simulink model "Automotive_model2"  (R2020b)
settings: Solver=VariableStepAuto  StartTime=0.0  StopTime=97  RelTol=1e-3
undefined symbols (not defined in the file): sigbuilder_block
libraries: simulink x23
(part 1 of 2)
settings Model: Creator=99003757  LastModifiedBy=99003727
settings OptimizationCC: DefaultUnderspecifiedDataType=single
settings DebuggingCC: UniqueDataStoreMsg=error
settings ConfigComp: CovEnable=on  CovScope=ReferencedModels  CovIncludeTopModel=off  CovMetricSettings=dcmwe  CovModelRefEnable=on

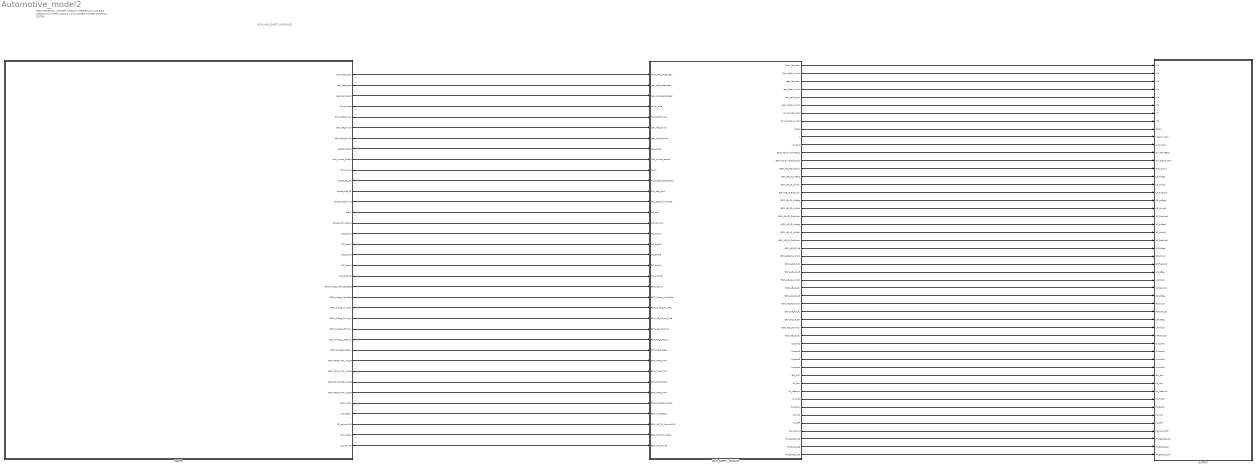
== system Automotive_model2 ==
  note: REQUIREMENTS:
      |
      | 1.POWER WINDOW OPEARTION
      | 2.AIR BAG OPEARTION
      | 3.TPMS
      | 4.DOOR LOCK SYSTEM
      | 5.WIPER CONTROL SYSTEM
  note: BCM_AND_SAFETY_MODULES
  BCM_SAFETY_MODULE : Subsystem
  INPUTS : Subsystem
  OUTPUT : Subsystem
  wires:
  INPUTS/1(Front_left_pass) -> BCM_SAFETY_MODULE/1(Front_left_passenger)
  INPUTS/2(rear_left_pass) -> BCM_SAFETY_MODULE/2(rear_left_passenger)
  INPUTS/3(rear_right_pass) -> BCM_SAFETY_MODULE/3(rear_right_passenger)
  INPUTS/4(Driver_side) -> BCM_SAFETY_MODULE/4(driver_side)
  INPUTS/5(Front_left_driver) -> BCM_SAFETY_MODULE/5(front_left_driver)
  INPUTS/6(rear_left_driver) -> BCM_SAFETY_MODULE/6(rear_left_driver)
  INPUTS/7(rear_right_driver) -> BCM_SAFETY_MODULE/7(rear_right_driver)
  INPUTS/8(object_det_FL) -> BCM_SAFETY_MODULE/8(object_res)
  INPUTS/9(lock_unlock_button) -> BCM_SAFETY_MODULE/9(lock_unlock_control)
  INPUTS/10(ignition_sw) -> BCM_SAFETY_MODULE/10(Ig_sw)
  INPUTS/11(object_det_RL) -> BCM_SAFETY_MODULE/11(Right_left_object_detc)
  INPUTS/12(object_det_RR) -> BCM_SAFETY_MODULE/12(Obj_det_right)
  INPUTS/13(object_det_driver) -> BCM_SAFETY_MODULE/13(Obj_Detc_driver-side)
  INPUTS/14(accln) -> BCM_SAFETY_MODULE/14(DC_Acc)
  INPUTS/15(DC_ignition_status) -> BCM_SAFETY_MODULE/15(DC_iginition)
  INPUTS/16(DC_Door1) -> BCM_SAFETY_MODULE/16(DC_Door1)
  INPUTS/17(DC_Door2) -> BCM_SAFETY_MODULE/17(DC_Door2)
  INPUTS/18(DC_Door3) -> BCM_SAFETY_MODULE/18(DC_Door3)
  INPUTS/19(DC_Door4) -> BCM_SAFETY_MODULE/19(DC_Door4)
  INPUTS/20(DC_antilock) -> BCM_SAFETY_MODULE/20(DC_Antilock)
  INPUTS/21(BAM_Airbag_VehicleSpeed) -> BCM_SAFETY_MODULE/21(BCM_AB_VS)
  INPUTS/22(BCM_Airbag_YawRate) -> BCM_SAFETY_MODULE/22(BCM_Airbag_YawRate)
  INPUTS/23(BCM_Airbag_Air_ACC) -> BCM_SAFETY_MODULE/23(BCM_Airbag_Air_ACC)
  INPUTS/24(BCM_Airbag_Driver_L) -> BCM_SAFETY_MODULE/24(BCM_AB_Driver_Side)
  INPUTS/25(BCM_AirbagL_Front_1) -> BCM_SAFETY_MODULE/25(BCM_AB_L_Front_1)
  INPUTS/26(BCM_Airbag_L_Rear_1) -> BCM_SAFETY_MODULE/26(BCM_AB_L_Rear_1)
  INPUTS/27(BCM_Airbag_R_Rear_) -> BCM_SAFETY_MODULE/27(BCM_AB_R_Rear_)
  BCM_SAFETY_MODULE/1(Front_left_warn) -> OUTPUT/1(In1)
  BCM_SAFETY_MODULE/2(Front_left_window) -> OUTPUT/2(In2)
  BCM_SAFETY_MODULE/3(rear_left_warn) -> OUTPUT/3(In3)
  BCM_SAFETY_MODULE/4(rear_left_window) -> OUTPUT/4(In4)
  BCM_SAFETY_MODULE/5(rear_right_warn) -> OUTPUT/5(In5)
  BCM_SAFETY_MODULE/6(rear_right_window) -> OUTPUT/6(In6)
  BCM_SAFETY_MODULE/7(driver_side_warn) -> OUTPUT/7(In7)
  BCM_SAFETY_MODULE/8(driver_side_window) -> OUTPUT/8(In8)
  BCM_SAFETY_MODULE/9(Delay) -> OUTPUT/9(Delay)
  BCM_SAFETY_MODULE/10(y) -> OUTPUT/10(Interior light)
  BCM_SAFETY_MODULE/11(Outport) -> OUTPUT/11(Automatic)
  BCM_SAFETY_MODULE/12(BCM_AB_DriverAirBag1) -> OUTPUT/12(DriverAirBag1)
  BCM_SAFETY_MODULE/13(BCM_AB_DriverDoorLock) -> OUTPUT/13(DriverDoorLock)
  BCM_SAFETY_MODULE/14(BCM_AB_FuelLock11) -> OUTPUT/14(FuelLock11)
  BCM_SAFETY_MODULE/15(BCM_AB_LF_AirBag) -> OUTPUT/15(LF_AirBag)
  BCM_SAFETY_MODULE/16(BCM_AB_LF_Unlock) -> OUTPUT/16(LF_Unlock)
  BCM_SAFETY_MODULE/17(BCM_AB_LF_FuelLock) -> OUTPUT/17(LF_FuleLock)
  BCM_SAFETY_MODULE/18(BCM_AB_RR_AirBag) -> OUTPUT/18(RR_AirBag)
  BCM_SAFETY_MODULE/19(BCM_AB_RR_Unlock) -> OUTPUT/19(RR_Unlock)
  BCM_SAFETY_MODULE/20(BCM_AB_RR_FuelLock) -> OUTPUT/20(RR_FuelLock)
  BCM_SAFETY_MODULE/21(BCM_AB_LR_AirBag) -> OUTPUT/21(LR_AirBag)
  BCM_SAFETY_MODULE/22(BCM_AB_LR_Unlock) -> OUTPUT/22(LR_Unlock)
  BCM_SAFETY_MODULE/23(BCM_AB_LR_FuelLock) -> OUTPUT/23(LR_FuelLock)
  BCM_SAFETY_MODULE/24(BCM_AB_DS_AB) -> OUTPUT/24(DSAirBag)
  BCM_SAFETY_MODULE/25(BCM_AB_DS_Unlock) -> OUTPUT/25(DSUnlock)
  BCM_SAFETY_MODULE/26(BCM_AB_DS_FL) -> OUTPUT/26(DSFuelLock)
  BCM_SAFETY_MODULE/27(BCM_AB_LS_AB) -> OUTPUT/27(LSAirBag)
  BCM_SAFETY_MODULE/28(BCM_AB_LS_Unlock) -> OUTPUT/28(LSUnlock)
  BCM_SAFETY_MODULE/29(BCM_AB_LS_FL) -> OUTPUT/29(LSFuelLock)
  BCM_SAFETY_MODULE/30(BCM_AB_RS_AB) -> OUTPUT/30(RSAirBag)
  BCM_SAFETY_MODULE/31(BCM_AB_RSUnlock) -> OUTPUT/31(RSUnlock)
  BCM_SAFETY_MODULE/32(BCM_AB_RS_FL) -> OUTPUT/32(RSFuelLock)
  BCM_SAFETY_MODULE/33(BCM_AB_LR_AB) -> OUTPUT/33(LRAirBag)
  BCM_SAFETY_MODULE/34(BCM_AB_LRUnlock) -> OUTPUT/34(LRUnlock)
  BCM_SAFETY_MODULE/35(BCM_AB_LR_FL) -> OUTPUT/35(LRFuelLock)
  BCM_SAFETY_MODULE/36(Outport1) -> OUTPUT/36(Outport1)
  BCM_SAFETY_MODULE/37(Outport2) -> OUTPUT/37(Outport2)
  BCM_SAFETY_MODULE/38(Outport3) -> OUTPUT/38(Outport3)
  BCM_SAFETY_MODULE/39(Outport4) -> OUTPUT/39(Outport4)
  INPUTS/28(BCM_TPMS_TP1_VALUE) -> BCM_SAFETY_MODULE/28(BCM_TPMS_TP1)
  INPUTS/29(BCM_TPMS_TP2_VALUE) -> BCM_SAFETY_MODULE/29(BCM_TPMS_TP2)
  INPUTS/30(BCM_TPMS_TP3_VALUE) -> BCM_SAFETY_MODULE/30(BCM_TPMS_TP3)
  INPUTS/31(BCM_TPMS_TP4_VALUE) -> BCM_SAFETY_MODULE/31(BCM_TPMS_TP4)
  INPUTS/32(Rear_wiper) -> BCM_SAFETY_MODULE/32(BCM_WC_Rear_Wiper)
  INPUTS/33(WC_status) -> BCM_SAFETY_MODULE/33(BCM_WC_Status)
  INPUTS/34(FC_manualINP) -> BCM_SAFETY_MODULE/34(BCM_WC_FR_ManualINP)
  INPUTS/35(FW_Modes) -> BCM_SAFETY_MODULE/35(BCM_WC_FW_Modes)
  INPUTS/36(WC_FrontS) -> BCM_SAFETY_MODULE/36(BCM_WC_FrontS)
  BCM_SAFETY_MODULE/40(BW_OUT) -> OUTPUT/40(BW_out)
  BCM_SAFETY_MODULE/41(FA_Low) -> OUTPUT/41(FA_Low)
  BCM_SAFETY_MODULE/42(FA_Medium) -> OUTPUT/42(FA_Medium)
  BCM_SAFETY_MODULE/43(FA_High) -> OUTPUT/43(FA_HIGH)
  BCM_SAFETY_MODULE/44(FA_Spray) -> OUTPUT/44(FA_Spray)
  BCM_SAFETY_MODULE/45(FA_Mist) -> OUTPUT/45(FA_Mist)
  BCM_SAFETY_MODULE/46(FA_OFF) -> OUTPUT/46(FA_OFF)
  BCM_SAFETY_MODULE/47(Manual_out) -> OUTPUT/47(Manual_OUT)
  BCM_SAFETY_MODULE/48(FM_lessthan30) -> OUTPUT/48(FM_lessthan30)
  BCM_SAFETY_MODULE/49(FM_Bw30_60) -> OUTPUT/49(FM_Bw30_60)
  BCM_SAFETY_MODULE/50(FM_Bw60_100) -> OUTPUT/50(FM_Bw60_100)

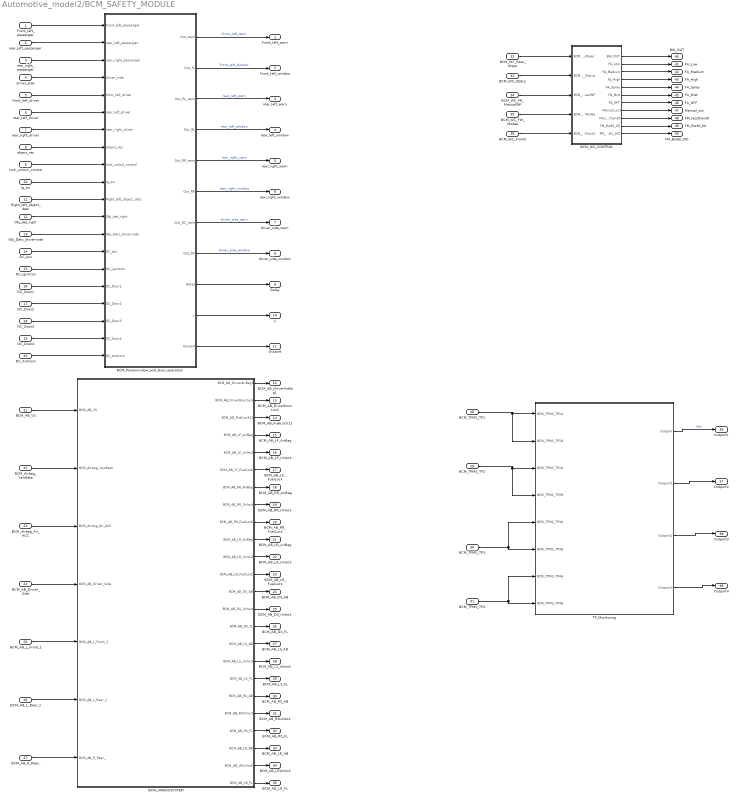
== system Automotive_model2/BCM_SAFETY_MODULE ==
  Front_left_passenger : Inport
  rear_left_passenger : Inport  Port=2
  rear_right_passenger : Inport  Port=3
  driver_side : Inport  Port=4
  front_left_driver : Inport  Port=5
  rear_left_driver : Inport  Port=6
  rear_right_driver : Inport  Port=7
  object_res : Inport  Port=8
  lock_unlock_control : Inport  Port=9
  Ig_sw : Inport  Port=10
  Right_left_object_detc : Inport  Port=11
  Obj_det_right : Inport  Port=12
  Obj_Detc_driver-side : Inport  Port=13
  DC_Acc : Inport  Port=14
  DC_iginition : Inport  Port=15
  DC_Door1 : Inport  Port=16
  DC_Door2 : Inport  Port=17
  DC_Door3 : Inport  Port=18
  DC_Door4 : Inport  Port=19
  DC_Antilock : Inport  Port=20
  BCM_AB_VS : Inport  Port=21
  BCM_Airbag_YawRate : Inport  Port=22
  BCM_Airbag_Air_ACC : Inport  Port=23
  BCM_AB_Driver_Side : Inport  Port=24
  BCM_AB_L_Front_1 : Inport  Port=25
  BCM_AB_L_Rear_1 : Inport  Port=26
  BCM_AB_R_Rear_ : Inport  Port=27
  BCM_TPMS_TP1 : Inport  Port=28
  BCM_TPMS_TP2 : Inport  Port=29
  BCM_TPMS_TP3 : Inport  Port=30
  BCM_TPMS_TP4 : Inport  Port=31
  BCM_WC_Rear_Wiper : Inport  Port=32
  BCM_WC_Status : Inport  Port=33
  BCM_WC_FR_ManualINP : Inport  Port=34
  BCM_WC_FW_Modes : Inport  Port=35
  BCM_WC_FrontS : Inport  Port=36
  BCM_AIRBAGSYSTEM : Subsystem
  BCM_Powerwindow_and_Door_operation : Subsystem
  BCM_WC_CONTROL : Subsystem
  TP_Monitoring : Subsystem
  Front_left_warn : Outport
  Front_left_window : Outport  Port=2
  rear_left_warn : Outport  Port=3
  rear_left_window : Outport  Port=4
  rear_right_warn : Outport  Port=5
  rear_right_window : Outport  Port=6
  driver_side_warn : Outport  Port=7
  driver_side_window : Outport  Port=8
  Delay : Outport  Port=9
  y : Outport  Port=10
  Outport : Outport  Port=11
  BCM_AB_DriverAirBag1 : Outport  Port=12
  BCM_AB_DriverDoorLock : Outport  Port=13
  BCM_AB_FuelLock11 : Outport  Port=14
  BCM_AB_LF_AirBag : Outport  Port=15
  BCM_AB_LF_Unlock : Outport  Port=16
  BCM_AB_LF_FuelLock : Outport  Port=17
  BCM_AB_RR_AirBag : Outport  Port=18
  BCM_AB_RR_Unlock : Outport  Port=19
  BCM_AB_RR_FuelLock : Outport  Port=20
  BCM_AB_LR_AirBag : Outport  Port=21
  BCM_AB_LR_Unlock : Outport  Port=22
  BCM_AB_LR_FuelLock : Outport  Port=23
  BCM_AB_DS_AB : Outport  Port=24
  BCM_AB_DS_Unlock : Outport  Port=25
  BCM_AB_DS_FL : Outport  Port=26
  BCM_AB_LS_AB : Outport  Port=27
  BCM_AB_LS_Unlock : Outport  Port=28
  BCM_AB_LS_FL : Outport  Port=29
  BCM_AB_RS_AB : Outport  Port=30
  BCM_AB_RSUnlock : Outport  Port=31
  BCM_AB_RS_FL : Outport  Port=32
  BCM_AB_LR_AB : Outport  Port=33
  BCM_AB_LRUnlock : Outport  Port=34
  BCM_AB_LR_FL : Outport  Port=35
  Outport1 : Outport  Port=36
  Outport2 : Outport  Port=37
  Outport3 : Outport  Port=38
  Outport4 : Outport  Port=39
  BW_OUT : Outport  Port=40
  FA_Low : Outport  Port=41
  FA_Medium : Outport  Port=42
  FA_High : Outport  Port=43
  FA_Spray : Outport  Port=44
  FA_Mist : Outport  Port=45
  FA_OFF : Outport  Port=46
  Manual_out : Outport  Port=47
  FM_lessthan30 : Outport  Port=48
  FM_Bw30_60 : Outport  Port=49
  FM_Bw60_100 : Outport  Port=50
  wires:
  BCM_Powerwindow_and_Door_operation/5(Out_RR_warn) -> rear_right_warn/1  "rear_right_warn"
  BCM_AB_VS/1 -> BCM_AIRBAGSYSTEM/1(BCM_AB_VS)
  BCM_Powerwindow_and_Door_operation/4(Out_RL) -> rear_left_window/1  "rear_left_window"
  BCM_AIRBAGSYSTEM/22(BCM_AB_LR_AB) -> BCM_AB_LR_AB/1
  BCM_AIRBAGSYSTEM/18(BCM_AB_LS_FL) -> BCM_AB_LS_FL/1
  BCM_AIRBAGSYSTEM/10(BCM_AB_LR_AirBag) -> BCM_AB_LR_AirBag/1
  BCM_AIRBAGSYSTEM/11(BCM_AB_LR_Unlock) -> BCM_AB_LR_Unlock/1
  BCM_Powerwindow_and_Door_operation/10(y) -> y/1
  BCM_Powerwindow_and_Door_operation/9(Delay) -> Delay/1
  BCM_Powerwindow_and_Door_operation/7(Out_DC_warn) -> driver_side_warn/1  "driver_side_warn"
  DC_Door2/1 -> BCM_Powerwindow_and_Door_operation/17(DC_Door2)
  BCM_AB_R_Rear_/1 -> BCM_AIRBAGSYSTEM/7(BCM_AB_R_Rear_)
  DC_Door1/1 -> BCM_Powerwindow_and_Door_operation/16(DC_Door1)
  DC_Door3/1 -> BCM_Powerwindow_and_Door_operation/18(DC_Door3)
  BCM_AIRBAGSYSTEM/23(BCM_AB_LRUnlock) -> BCM_AB_LRUnlock/1
  BCM_AIRBAGSYSTEM/24(BCM_AB_LR_FL) -> BCM_AB_LR_FL/1
  BCM_AIRBAGSYSTEM/9(BCM_AB_RR_FuelLock) -> BCM_AB_RR_FuelLock/1
  BCM_AIRBAGSYSTEM/17(BCM_AB_LS_Unlock) -> BCM_AB_LS_Unlock/1
  BCM_Powerwindow_and_Door_operation/6(Out_RR) -> rear_right_window/1  "rear_right_window"
  BCM_Powerwindow_and_Door_operation/1(Out_warn) -> Front_left_warn/1  "Front_left_warn"
  BCM_Powerwindow_and_Door_operation/8(Out_DC) -> driver_side_window/1  "driver_side_window"
  BCM_Powerwindow_and_Door_operation/2(Out_FL) -> Front_left_window/1  "Front_left_window"
  rear_right_driver/1 -> BCM_Powerwindow_and_Door_operation/7(rear_right_driver)
  BCM_Powerwindow_and_Door_operation/11(Outport) -> Outport/1
  Ig_sw/1 -> BCM_Powerwindow_and_Door_operation/10(Ig_sw)
  object_res/1 -> BCM_Powerwindow_and_Door_operation/8(object_res)
  lock_unlock_control/1 -> BCM_Powerwindow_and_Door_operation/9(lock_unlock_control)
  rear_left_passenger/1 -> BCM_Powerwindow_and_Door_operation/2(rear_left_passenger)
  DC_iginition/1 -> BCM_Powerwindow_and_Door_operation/15(DC_iginition)
  DC_Antilock/1 -> BCM_Powerwindow_and_Door_operation/20(DC_Antilock)
  BCM_Powerwindow_and_Door_operation/3(Out_RL_warn) -> rear_left_warn/1  "rear_left_warn"
  DC_Acc/1 -> BCM_Powerwindow_and_Door_operation/14(DC_Acc)
  BCM_AIRBAGSYSTEM/15(BCM_AB_DS_FL) -> BCM_AB_DS_FL/1
  BCM_AIRBAGSYSTEM/3(BCM_AB_FuelLock11) -> BCM_AB_FuelLock11/1
  BCM_AIRBAGSYSTEM/7(BCM_AB_RR_AirBag) -> BCM_AB_RR_AirBag/1
  BCM_AIRBAGSYSTEM/4(BCM_AB_LF_AirBag) -> BCM_AB_LF_AirBag/1
  BCM_AIRBAGSYSTEM/13(BCM_AB_DS_AB) -> BCM_AB_DS_AB/1
  Obj_det_right/1 -> BCM_Powerwindow_and_Door_operation/12(Obj_det_right)
  Obj_Detc_driver-side/1 -> BCM_Powerwindow_and_Door_operation/13(Obj_Detc_driver-side)
  rear_right_passenger/1 -> BCM_Powerwindow_and_Door_operation/3(rear_right_passenger)
  Right_left_object_detc/1 -> BCM_Powerwindow_and_Door_operation/11(Right_left_object_detc)
  driver_side/1 -> BCM_Powerwindow_and_Door_operation/4(driver_side)
  rear_left_driver/1 -> BCM_Powerwindow_and_Door_operation/6(rear_left_driver)
  front_left_driver/1 -> BCM_Powerwindow_and_Door_operation/5(front_left_driver)
  Front_left_passenger/1 -> BCM_Powerwindow_and_Door_operation/1(Front_left_passenger)
  BCM_AIRBAGSYSTEM/1(BCM_AB_DriverAirBag1) -> BCM_AB_DriverAirBag1/1
  BCM_AIRBAGSYSTEM/5(BCM_AB_LF_Unlock) -> BCM_AB_LF_Unlock/1
  BCM_AIRBAGSYSTEM/8(BCM_AB_RR_Unlock) -> BCM_AB_RR_Unlock/1
  BCM_AIRBAGSYSTEM/21(BCM_AB_RS_FL) -> BCM_AB_RS_FL/1
  BCM_AIRBAGSYSTEM/20(BCM_AB_RSUnlock) -> BCM_AB_RSUnlock/1
  BCM_AIRBAGSYSTEM/12(BCM_AB_LR_FuelLock) -> BCM_AB_LR_FuelLock/1
  BCM_AIRBAGSYSTEM/19(BCM_AB_RS_AB) -> BCM_AB_RS_AB/1
  BCM_AIRBAGSYSTEM/16(BCM_AB_LS_AB) -> BCM_AB_LS_AB/1
  BCM_AIRBAGSYSTEM/2(BCM_AB_DriverDoorLock) -> BCM_AB_DriverDoorLock/1
  BCM_AIRBAGSYSTEM/6(BCM_AB_LF_FuelLock) -> BCM_AB_LF_FuelLock/1
  BCM_AB_L_Rear_1/1 -> BCM_AIRBAGSYSTEM/6(BCM_AB_L_Rear_1)
  DC_Door4/1 -> BCM_Powerwindow_and_Door_operation/19(DC_Door4)
  BCM_AIRBAGSYSTEM/14(BCM_AB_DS_Unlock) -> BCM_AB_DS_Unlock/1
  BCM_AB_L_Front_1/1 -> BCM_AIRBAGSYSTEM/5(BCM_AB_L_Front_1)
  TP_Monitoring/1(Outport) -> Outport1/1  "op1"
  BCM_AB_Driver_Side/1 -> BCM_AIRBAGSYSTEM/4(BCM_AB_Driver_Side)
  BCM_Airbag_YawRate/1 -> BCM_AIRBAGSYSTEM/2(BCM_Airbag_YawRate)
  BCM_Airbag_Air_ACC/1 -> BCM_AIRBAGSYSTEM/3(BCM_Airbag_Air_ACC)
  TP_Monitoring/3(Outport2) -> Outport3/1
  TP_Monitoring/4(Outport3) -> Outport4/1
  TP_Monitoring/2(Outport1) -> Outport2/1
  BCM_TPMS_TP4/1 -> TP_Monitoring/8(BCM_TPMS_TP4B), TP_Monitoring/7(BCM_TPMS_TP4A)
  BCM_TPMS_TP2/1 -> TP_Monitoring/4(BCM_TPMS_TP2B), TP_Monitoring/3(BCM_TPMS_TP2A)
  BCM_TPMS_TP1/1 -> TP_Monitoring/2(BCM_TPMS_TP1B), TP_Monitoring/1(BCM_TPMS_TP1A)
  BCM_TPMS_TP3/1 -> TP_Monitoring/6(BCM_TPMS_TP3B), TP_Monitoring/5(BCM_TPMS_TP3A)
  BCM_WC_CONTROL/7(FA_OFF) -> FA_OFF/1
  BCM_WC_CONTROL/4(FA_High) -> FA_High/1
  BCM_WC_CONTROL/3(FA_Medium) -> FA_Medium/1
  BCM_WC_CONTROL/2(FA_Low) -> FA_Low/1
  BCM_WC_CONTROL/11(FM_Bw60_100) -> FM_Bw60_100/1
  BCM_WC_FrontS/1 -> BCM_WC_CONTROL/5(BCM_WC_FrontS)
  BCM_WC_Rear_Wiper/1 -> BCM_WC_CONTROL/1(BCM_WC_Rear_Wiper)
  BCM_WC_CONTROL/5(FA_Spray) -> FA_Spray/1
  BCM_WC_FW_Modes/1 -> BCM_WC_CONTROL/4(BCM_WC_FW_Modes)
  BCM_WC_CONTROL/9(FM_lessthan30) -> FM_lessthan30/1
  BCM_WC_FR_ManualINP/1 -> BCM_WC_CONTROL/3(BCM_WC_FR_ManualINP)
  BCM_WC_CONTROL/1(BW_OUT) -> BW_OUT/1
  BCM_WC_CONTROL/10(FM_Bw30_60) -> FM_Bw30_60/1
  BCM_WC_CONTROL/6(FA_Mist) -> FA_Mist/1
  BCM_WC_Status/1 -> BCM_WC_CONTROL/2(BCM_WC_Status)
  BCM_WC_CONTROL/8(Manual_out) -> Manual_out/1

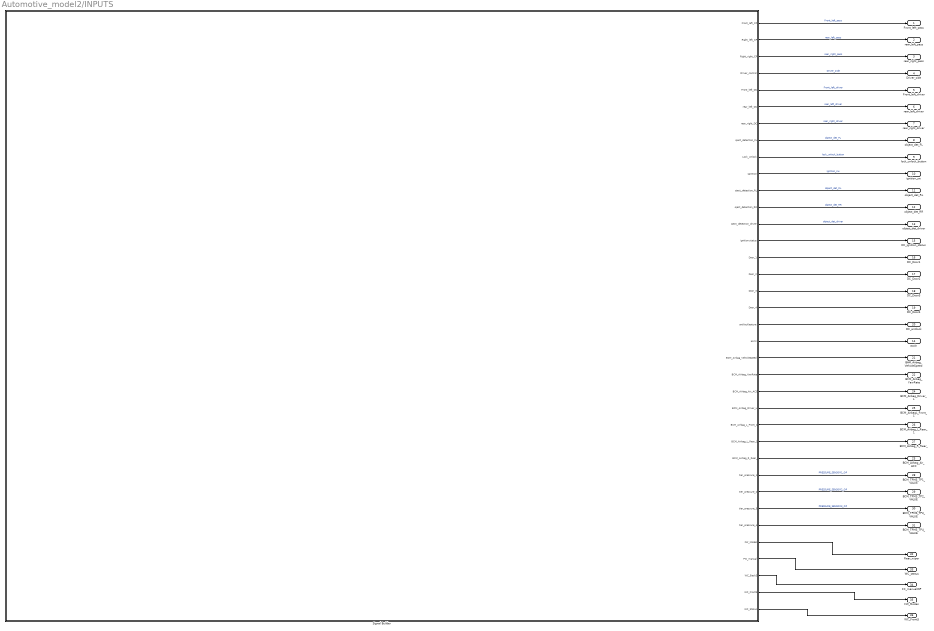
== system Automotive_model2/INPUTS ==
  Signal Builder : Subsystem  Tag=STV Subsys  LoadFcn=sigbuilder_block('load');  StartFcn=sigbuilder_block('start');  StopFcn=sigbuilder_block('stop');  ClipboardFcn=sigbuilder_block('clipboard');  mask(Sigbuilder block){tuvar=[0:10]}
      mask help: Simulink:masks:SigbuilderBlock_MD
      mask init:
      | if ~strcmp(get_param(bdroot(gcbh),'SimulationStatus'),'stopped') tuvar = sigbuilder_block('maskInit'); end
      settings: CopyFcn=sigbuilder_block('copy');  DeleteFcn=sigbuilder_block('delete');  ModelCloseFcn=sigbuilder_block('modelClose');  PreSaveFcn=sigbuilder_block('preSave');  PauseFcn=sigbuilder_block('pause');  ContinueFcn=sigbuilder_block('continue');  NameChangeFcn=sigbuilder_block('namechange');  OpenFcn=sigbuilder_block('open',[6 30 1188 546.75 ]);  CloseFcn=sigbuilder_block('close');
      mask Display: plot(0, 0, 100, 100,[2, 2, 32, 32, 2], [68, 8, 8, 68, 68],[32, 2], [38, 38], [32, 19, 2],[53, 60, 44], [32, 17, 17, 2],[16, 16, 31, 31]);txt = getActiveGroup(gcbh);text(2, 100, txt,'verticalAlignment', 'top');
  Front_left_pass : Outport
  rear_left_pass : Outport  Port=2
  rear_right_pass : Outport  Port=3
  Driver_side : Outport  Port=4
  Front_left_driver : Outport  Port=5
  rear_left_driver : Outport  Port=6
  rear_right_driver : Outport  Port=7
  object_det_FL : Outport  Port=8
  lock_unlock_button : Outport  Port=9
  ignition_sw : Outport  Port=10
  object_det_RL : Outport  Port=11
  object_det_RR : Outport  Port=12
  object_det_driver : Outport  Port=13
  accln : Outport  Port=14
  DC_ignition_status : Outport  Port=15
  DC_Door1 : Outport  Port=16
  DC_Door2 : Outport  Port=17
  DC_Door3 : Outport  Port=18
  DC_Door4 : Outport  Port=19
  DC_antilock : Outport  Port=20
  BAM_Airbag_VehicleSpeed : Outport  Port=21
  BCM_Airbag_YawRate : Outport  Port=22
  BCM_Airbag_Air_ACC : Outport  Port=23
  BCM_Airbag_Driver_L : Outport  Port=24
  BCM_AirbagL_Front_1 : Outport  Port=25
  BCM_Airbag_L_Rear_1 : Outport  Port=26
  BCM_Airbag_R_Rear_ : Outport  Port=27
  BCM_TPMS_TP1_VALUE : Outport  Port=28
  BCM_TPMS_TP2_VALUE : Outport  Port=29
  BCM_TPMS_TP3_VALUE : Outport  Port=30
  BCM_TPMS_TP4_VALUE : Outport  Port=31
  Rear_wiper : Outport  Port=32
  WC_status : Outport  Port=33
  FC_manualINP : Outport  Port=34
  FW_Modes : Outport  Port=35
  WC_FrontS : Outport  Port=36
  wires:
  Signal Builder/14(ignition status) -> DC_ignition_status/1
  Signal Builder/25(BCM_Airbag_L_Front_1) -> BCM_Airbag_L_Rear_1/1
  Signal Builder/21(BCM_Airbag_VehicleSpeed) -> BAM_Airbag_VehicleSpeed/1
  Signal Builder/22(BCM_Airbag_YawRate) -> BCM_Airbag_YawRate/1
  Signal Builder/11(oject_detection_RL) -> object_det_RL/1  "object_det_RL"
  Signal Builder/12(oject_detection_RR) -> object_det_RR/1  "object_det_RR"
  Signal Builder/27(BCM_Airbag_R_Rear_) -> BCM_Airbag_Air_ACC/1
  Signal Builder/26(BCM_Airbag_L_Rear_1) -> BCM_Airbag_R_Rear_/1
  Signal Builder/24(BCM_Airbag_Driver_L) -> BCM_AirbagL_Front_1/1
  Signal Builder/23(BCM_Airbag_Air_ACC) -> BCM_Airbag_Driver_L/1
  Signal Builder/20(accln) -> accln/1
  Signal Builder/19(antilockleature) -> DC_antilock/1
  Signal Builder/2(Right_left_CP) -> rear_left_pass/1  "rear_left_pass"
  Signal Builder/3(Right_right_CP) -> rear_right_pass/1  "rear_right_pass"
  Signal Builder/18(Door_4) -> DC_Door4/1
  Signal Builder/17(Door_3) -> DC_Door3/1
  Signal Builder/16(Door_2) -> DC_Door2/1
  Signal Builder/15(Door_1) -> DC_Door1/1
  Signal Builder/30(tier_pressure_3) -> BCM_TPMS_TP3_VALUE/1  "PRESSURE_SENSOR3_OP"
  Signal Builder/29(tier_pressure_2) -> BCM_TPMS_TP2_VALUE/1  "PRESSURE_SENSOR2_OP"
  Signal Builder/28(tier_pressure_1) -> BCM_TPMS_TP1_VALUE/1  "PRESSURE_SENSOR1_OP"
  Signal Builder/13(oject_detection_driver) -> object_det_driver/1  "object_det_driver"
  Signal Builder/4(Driver_control) -> Driver_side/1  "Driver_side"
  Signal Builder/8(oject_detection_FL) -> object_det_FL/1  "object_det_FL"
  Signal Builder/5(Front_left_DC) -> Front_left_driver/1  "Front_left_driver"
  Signal Builder/7(rear_right_DC) -> rear_right_driver/1  "rear_right_driver"
  Signal Builder/10(iginition) -> ignition_sw/1  "ignition_sw"
  Signal Builder/1(Front_left_CP) -> Front_left_pass/1  "Front_left_pass"
  Signal Builder/6(rear_left_DC) -> rear_left_driver/1  "rear_left_driver"
  Signal Builder/9(Lock_Unlock) -> lock_unlock_button/1  "lock_unlock_button"
  Signal Builder/31(tier_pressure_4) -> BCM_TPMS_TP4_VALUE/1
  Signal Builder/32(FW_Modes) -> Rear_wiper/1
  Signal Builder/33(FW_manual) -> WC_status/1
  Signal Builder/34(WC_BackS) -> FC_manualINP/1
  Signal Builder/35(WC_FrontS) -> FW_Modes/1
  Signal Builder/36(WC_Status) -> WC_FrontS/1

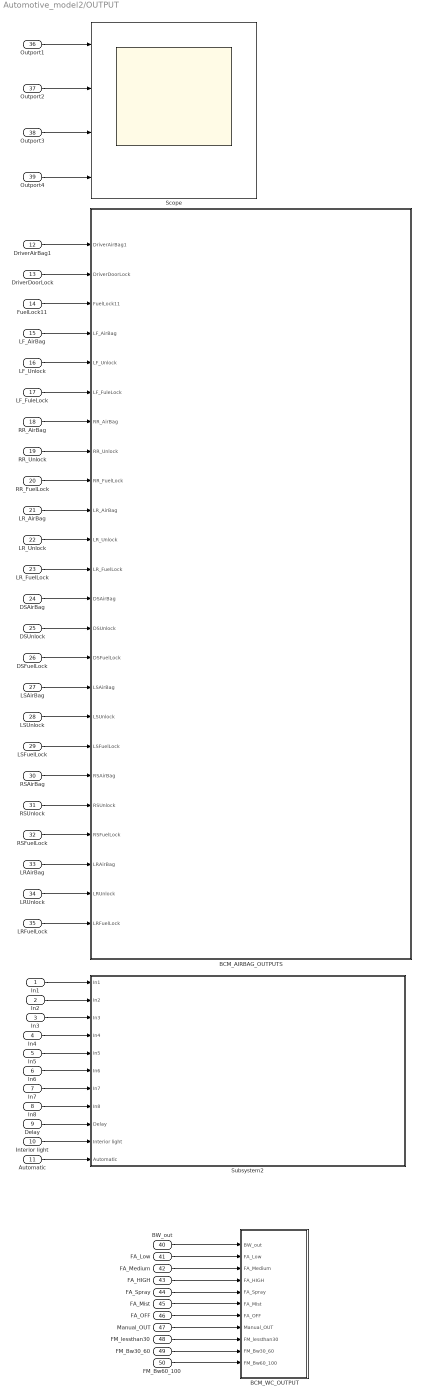
== system Automotive_model2/OUTPUT ==
  In1 : Inport
  In2 : Inport  Port=2
  In3 : Inport  Port=3
  In4 : Inport  Port=4
  In5 : Inport  Port=5
  In6 : Inport  Port=6
  In7 : Inport  Port=7
  In8 : Inport  Port=8
  Delay : Inport  Port=9
  Interior light : Inport  Port=10
  Automatic : Inport  Port=11
  DriverAirBag1 : Inport  Port=12
  DriverDoorLock : Inport  Port=13
  FuelLock11 : Inport  Port=14
  LF_AirBag : Inport  Port=15
  LF_Unlock : Inport  Port=16
  LF_FuleLock : Inport  Port=17
  RR_AirBag : Inport  Port=18
  RR_Unlock : Inport  Port=19
  RR_FuelLock : Inport  Port=20
  LR_AirBag : Inport  Port=21
  LR_Unlock : Inport  Port=22
  LR_FuelLock : Inport  Port=23
  DSAirBag : Inport  Port=24
  DSUnlock : Inport  Port=25
  DSFuelLock : Inport  Port=26
  LSAirBag : Inport  Port=27
  LSUnlock : Inport  Port=28
  LSFuelLock : Inport  Port=29
  RSAirBag : Inport  Port=30
  RSUnlock : Inport  Port=31
  RSFuelLock : Inport  Port=32
  LRAirBag : Inport  Port=33
  LRUnlock : Inport  Port=34
  LRFuelLock : Inport  Port=35
  Outport1 : Inport  Port=36
  Outport2 : Inport  Port=37
  Outport3 : Inport  Port=38
  Outport4 : Inport  Port=39
  BW_out : Inport  Port=40
  FA_Low : Inport  Port=41
  FA_Medium : Inport  Port=42
  FA_HIGH : Inport  Port=43
  FA_Spray : Inport  Port=44
  FA_Mist : Inport  Port=45
  FA_OFF : Inport  Port=46
  Manual_OUT : Inport  Port=47
  FM_lessthan30 : Inport  Port=48
  FM_Bw30_60 : Inport  Port=49
  FM_Bw60_100 : Inport  Port=50
  BCM_AIRBAG_OUTPUTS : Subsystem
  BCM_WC_OUTPUT : Subsystem
  Scope : Scope  NumInputPorts=4
  Subsystem2 : Subsystem
  wires:
  Outport1/1 -> Scope/1
  Outport4/1 -> Scope/4
  Outport3/1 -> Scope/3
  Outport2/1 -> Scope/2
  LSFuelLock/1 -> BCM_AIRBAG_OUTPUTS/18(LSFuelLock)
  RSAirBag/1 -> BCM_AIRBAG_OUTPUTS/19(RSAirBag)
  LRUnlock/1 -> BCM_AIRBAG_OUTPUTS/23(LRUnlock)
  LRAirBag/1 -> BCM_AIRBAG_OUTPUTS/22(LRAirBag)
  RR_FuelLock/1 -> BCM_AIRBAG_OUTPUTS/9(RR_FuelLock)
  LR_Unlock/1 -> BCM_AIRBAG_OUTPUTS/11(LR_Unlock)
  LSUnlock/1 -> BCM_AIRBAG_OUTPUTS/17(LSUnlock)
  LSAirBag/1 -> BCM_AIRBAG_OUTPUTS/16(LSAirBag)
  LR_FuelLock/1 -> BCM_AIRBAG_OUTPUTS/12(LR_FuelLock)
  LR_AirBag/1 -> BCM_AIRBAG_OUTPUTS/10(LR_AirBag)
  DSUnlock/1 -> BCM_AIRBAG_OUTPUTS/14(DSUnlock)
  DSAirBag/1 -> BCM_AIRBAG_OUTPUTS/13(DSAirBag)
  RSFuelLock/1 -> BCM_AIRBAG_OUTPUTS/21(RSFuelLock)
  RSUnlock/1 -> BCM_AIRBAG_OUTPUTS/20(RSUnlock)
  LRFuelLock/1 -> BCM_AIRBAG_OUTPUTS/24(LRFuelLock)
  DSFuelLock/1 -> BCM_AIRBAG_OUTPUTS/15(DSFuelLock)
  RR_AirBag/1 -> BCM_AIRBAG_OUTPUTS/7(RR_AirBag)
  LF_FuleLock/1 -> BCM_AIRBAG_OUTPUTS/6(LF_FuleLock)
  RR_Unlock/1 -> BCM_AIRBAG_OUTPUTS/8(RR_Unlock)
  In7/1 -> Subsystem2/7(In7)
  In4/1 -> Subsystem2/4(In4)
  LF_AirBag/1 -> BCM_AIRBAG_OUTPUTS/4(LF_AirBag)
  LF_Unlock/1 -> BCM_AIRBAG_OUTPUTS/5(LF_Unlock)
  FuelLock11/1 -> BCM_AIRBAG_OUTPUTS/3(FuelLock11)
  DriverAirBag1/1 -> BCM_AIRBAG_OUTPUTS/1(DriverAirBag1)
  Interior light/1 -> Subsystem2/10(Interior light)
  DriverDoorLock/1 -> BCM_AIRBAG_OUTPUTS/2(DriverDoorLock)
  Delay/1 -> Subsystem2/9(Delay)
  In6/1 -> Subsystem2/6(In6)
  Automatic/1 -> Subsystem2/11(Automatic)
  In8/1 -> Subsystem2/8(In8)
  In2/1 -> Subsystem2/2(In2)
  In5/1 -> Subsystem2/5(In5)
  In1/1 -> Subsystem2/1(In1)
  In3/1 -> Subsystem2/3(In3)
  FM_Bw60_100/1 -> BCM_WC_OUTPUT/11(FM_Bw60_100)
  FM_lessthan30/1 -> BCM_WC_OUTPUT/9(FM_lessthan30)
  FA_Mist/1 -> BCM_WC_OUTPUT/6(FA_Mist)
  FA_HIGH/1 -> BCM_WC_OUTPUT/4(FA_HIGH)
  FA_OFF/1 -> BCM_WC_OUTPUT/7(FA_OFF)
  FM_Bw30_60/1 -> BCM_WC_OUTPUT/10(FM_Bw30_60)
  FA_Low/1 -> BCM_WC_OUTPUT/2(FA_Low)
  Manual_OUT/1 -> BCM_WC_OUTPUT/8(Manual_OUT)
  FA_Medium/1 -> BCM_WC_OUTPUT/3(FA_Medium)
  BW_out/1 -> BCM_WC_OUTPUT/1(BW_out)
  FA_Spray/1 -> BCM_WC_OUTPUT/5(FA_Spray)

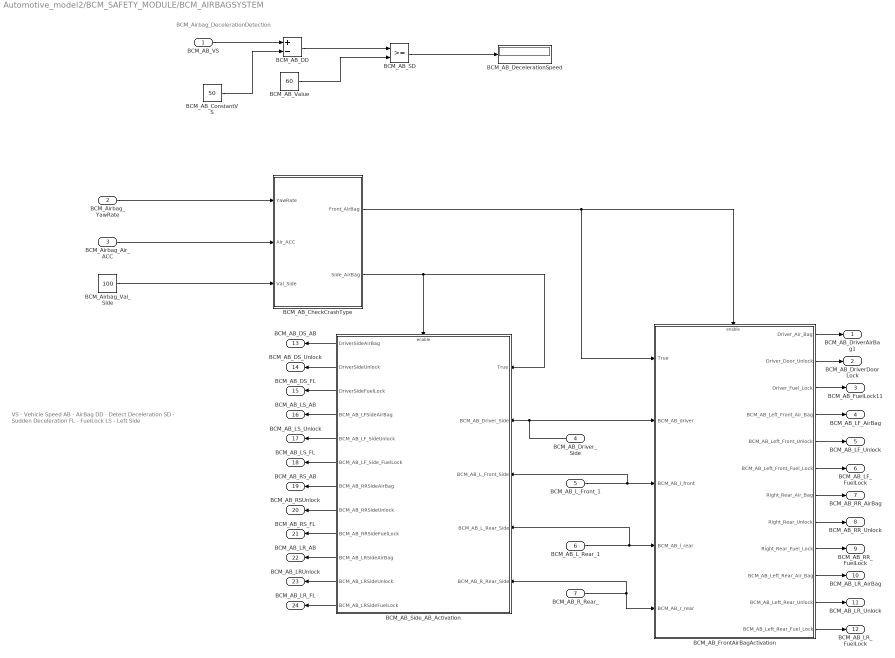
== system Automotive_model2/BCM_SAFETY_MODULE/BCM_AIRBAGSYSTEM ==
  note: VS - Vehicle Speed
      | AB - AirBag
      | DD - Detect Deceleration
      | SD - Sudden Deceleration
      | FL - FuelLock
      | LS - Left Side
  note: BCM_Airbag_DecelerationDetection
  BCM_AB_VS : Inport
  BCM_Airbag_YawRate : Inport  Port=2
  BCM_Airbag_Air_ACC : Inport  Port=3
  BCM_AB_Driver_Side : Inport  Port=4
  BCM_AB_L_Front_1 : Inport  Port=5
  BCM_AB_L_Rear_1 : Inport  Port=6
  BCM_AB_R_Rear_ : Inport  Port=7
  BCM_AB_CheckCrashType : Subsystem
  BCM_AB_ConstantVS : Constant  Value=50
  BCM_AB_DD : Sum  Inputs=+-
  BCM_AB_DecelerationSpeed : Display
  BCM_AB_FrontAirBagActivation : Subsystem  TreatAsAtomicUnit=on
  BCM_AB_SD : RelationalOperator  OutDataTypeStr=boolean  RndMeth=Simplest
  BCM_AB_Side_AB_Activation : Subsystem  TreatAsAtomicUnit=on
  BCM_AB_Value : Constant  Value=60
  BCM_Airbag_Val_Side : Constant  Value=100
  BCM_AB_DriverAirBag1 : Outport
  BCM_AB_DriverDoorLock : Outport  Port=2
  BCM_AB_FuelLock11 : Outport  Port=3
  BCM_AB_LF_AirBag : Outport  Port=4
  BCM_AB_LF_Unlock : Outport  Port=5
  BCM_AB_LF_FuelLock : Outport  Port=6
  BCM_AB_RR_AirBag : Outport  Port=7
  BCM_AB_RR_Unlock : Outport  Port=8
  BCM_AB_RR_FuelLock : Outport  Port=9
  BCM_AB_LR_AirBag : Outport  Port=10
  BCM_AB_LR_Unlock : Outport  Port=11
  BCM_AB_LR_FuelLock : Outport  Port=12
  BCM_AB_DS_AB : Outport  Port=13
  BCM_AB_DS_Unlock : Outport  Port=14
  BCM_AB_DS_FL : Outport  Port=15
  BCM_AB_LS_AB : Outport  Port=16
  BCM_AB_LS_Unlock : Outport  Port=17
  BCM_AB_LS_FL : Outport  Port=18
  BCM_AB_RS_AB : Outport  Port=19
  BCM_AB_RSUnlock : Outport  Port=20
  BCM_AB_RS_FL : Outport  Port=21
  BCM_AB_LR_AB : Outport  Port=22
  BCM_AB_LRUnlock : Outport  Port=23
  BCM_AB_LR_FL : Outport  Port=24
  wires:
  BCM_AB_ConstantVS/1 -> BCM_AB_DD/2
  BCM_AB_Value/1 -> BCM_AB_SD/2
  BCM_AB_DD/1 -> BCM_AB_SD/1
  BCM_AB_SD/1 -> BCM_AB_DecelerationSpeed/1
  BCM_AB_R_Rear_/1 -> BCM_AB_Side_AB_Activation/5(BCM_AB_R_Rear_Side), BCM_AB_FrontAirBagActivation/5(BCM_AB_r_rear)
  BCM_AB_L_Rear_1/1 -> BCM_AB_Side_AB_Activation/4(BCM_AB_L_Rear_Side), BCM_AB_FrontAirBagActivation/4(BCM_AB_l_rear)
  BCM_AB_VS/1 -> BCM_AB_DD/1
  BCM_AB_CheckCrashType/1(Front_AirBag) -> BCM_AB_FrontAirBagActivation/Enable, BCM_AB_FrontAirBagActivation/1(True)
  BCM_AB_CheckCrashType/2(Side_AirBag) -> BCM_AB_Side_AB_Activation/1(True), BCM_AB_Side_AB_Activation/Enable
  BCM_Airbag_YawRate/1 -> BCM_AB_CheckCrashType/1(YawRate)
  BCM_Airbag_Air_ACC/1 -> BCM_AB_CheckCrashType/2(Air_ACC)
  BCM_Airbag_Val_Side/1 -> BCM_AB_CheckCrashType/3(Val_Side)
  BCM_AB_Driver_Side/1 -> BCM_AB_Side_AB_Activation/2(BCM_AB_Driver_Side), BCM_AB_FrontAirBagActivation/2(BCM_AB_driver)
  BCM_AB_L_Front_1/1 -> BCM_AB_Side_AB_Activation/3(BCM_AB_L_Front_Side), BCM_AB_FrontAirBagActivation/3(BCM_AB_l_front)
  BCM_AB_Side_AB_Activation/2(DriverSideUnlock) -> BCM_AB_DS_Unlock/1
  BCM_AB_Side_AB_Activation/3(DriverSideFuelLock) -> BCM_AB_DS_FL/1
  BCM_AB_Side_AB_Activation/1(DriverSideAirBag) -> BCM_AB_DS_AB/1
  BCM_AB_Side_AB_Activation/12(BCM_AB_LRSideFuelLock) -> BCM_AB_LR_FL/1
  BCM_AB_Side_AB_Activation/11(BCM_AB_LRSideUnlock) -> BCM_AB_LRUnlock/1
  BCM_AB_Side_AB_Activation/10(BCM_AB_LRSideAirBag) -> BCM_AB_LR_AB/1
  BCM_AB_Side_AB_Activation/9(BCM_AB_RRSideFuelLock) -> BCM_AB_RS_FL/1
  BCM_AB_Side_AB_Activation/4(BCM_AB_LFSideAirBag) -> BCM_AB_LS_AB/1
  BCM_AB_Side_AB_Activation/5(BCM_AB_LF_SideUnlock) -> BCM_AB_LS_Unlock/1
  BCM_AB_Side_AB_Activation/6(BCM_AB_LF_Side_FuelLock) -> BCM_AB_LS_FL/1
  BCM_AB_Side_AB_Activation/7(BCM_AB_RRSideAirBag) -> BCM_AB_RS_AB/1
  BCM_AB_Side_AB_Activation/8(BCM_AB_RRSideUnlock) -> BCM_AB_RSUnlock/1
  BCM_AB_FrontAirBagActivation/12(BCM_AB_Left_Rear_Fuel_Lock) -> BCM_AB_LR_FuelLock/1
  BCM_AB_FrontAirBagActivation/11(BCM_AB_Left_Rear_Unlock) -> BCM_AB_LR_Unlock/1
  BCM_AB_FrontAirBagActivation/1(Driver_Air_Bag) -> BCM_AB_DriverAirBag1/1
  BCM_AB_FrontAirBagActivation/2(Driver_Door_Unlock) -> BCM_AB_DriverDoorLock/1
  BCM_AB_FrontAirBagActivation/3(Driver_Fuel_Lock) -> BCM_AB_FuelLock11/1
  BCM_AB_FrontAirBagActivation/4(BCM_AB_Left_Front_Air_Bag) -> BCM_AB_LF_AirBag/1
  BCM_AB_FrontAirBagActivation/5(BCM_AB_Left_Front_Unlock) -> BCM_AB_LF_Unlock/1
  BCM_AB_FrontAirBagActivation/6(BCM_AB_Left_Front_Fuel_Lock) -> BCM_AB_LF_FuelLock/1
  BCM_AB_FrontAirBagActivation/7(Right_Rear_Air_Bag) -> BCM_AB_RR_AirBag/1
  BCM_AB_FrontAirBagActivation/8(Right_Rear_Unlock) -> BCM_AB_RR_Unlock/1
  BCM_AB_FrontAirBagActivation/9(Right_Rear_Fuel_Lock) -> BCM_AB_RR_FuelLock/1
  BCM_AB_FrontAirBagActivation/10(BCM_AB_Left_Rear_Air_Bag) -> BCM_AB_LR_AirBag/1

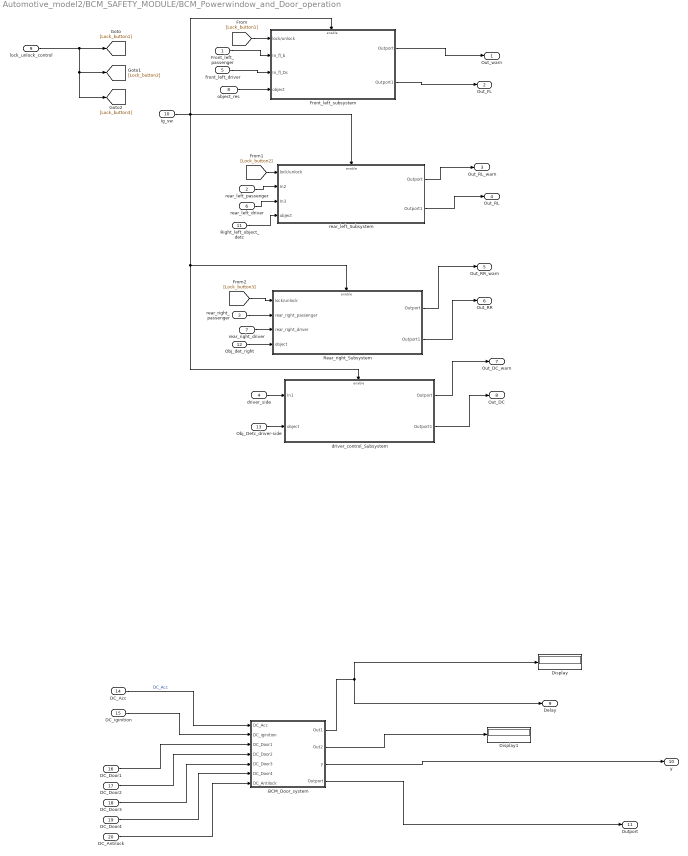
== system Automotive_model2/BCM_SAFETY_MODULE/BCM_Powerwindow_and_Door_operation ==
  Front_left_passenger : Inport
  rear_left_passenger : Inport  Port=2
  rear_right_passenger : Inport  Port=3
  driver_side : Inport  Port=4
  front_left_driver : Inport  Port=5
  rear_left_driver : Inport  Port=6
  rear_right_driver : Inport  Port=7
  object_res : Inport  Port=8
  lock_unlock_control : Inport  Port=9
  Ig_sw : Inport  Port=10
  Right_left_object_detc : Inport  Port=11
  Obj_det_right : Inport  Port=12
  Obj_Detc_driver-side : Inport  Port=13
  DC_Acc : Inport  Port=14
  DC_iginition : Inport  Port=15
  DC_Door1 : Inport  Port=16
  DC_Door2 : Inport  Port=17
  DC_Door3 : Inport  Port=18
  DC_Door4 : Inport  Port=19
  DC_Antilock : Inport  Port=20
  BCM_Door_system : Subsystem
  Display : Display
  Display1 : Display
  Front_left_subsystem : Subsystem
  Rear_right_Subsystem : Subsystem
  driver_control_Subsystem : Subsystem
  rear_left_Subsystem : Subsystem
  Out_warn : Outport
  Out_FL : Outport  Port=2
  Out_RL_warn : Outport  Port=3
  Out_RL : Outport  Port=4
  Out_RR_warn : Outport  Port=5
  Out_RR : Outport  Port=6
  Out_DC_warn : Outport  Port=7
  Out_DC : Outport  Port=8
  Delay : Outport  Port=9
  y : Outport  Port=10
  Outport : Outport  Port=11
  wires:
  Front_left_subsystem/1(Outport) -> Out_warn/1
  Front_left_subsystem/2(Outport1) -> Out_FL/1
  rear_left_Subsystem/1(Outport) -> Out_RL_warn/1
  rear_left_Subsystem/2(Outport1) -> Out_RL/1
  Rear_right_Subsystem/1(Outport) -> Out_RR_warn/1
  Rear_right_Subsystem/2(Outport1) -> Out_RR/1
  driver_control_Subsystem/1(Outport) -> Out_DC_warn/1
  driver_control_Subsystem/2(Outport1) -> Out_DC/1
  lock_unlock_control/1 -> [Lock_button3], [Lock_button2], [Lock_button1]
  front_left_driver/1 -> Front_left_subsystem/3(In_fl_Dc)
  [Lock_button1] -> Front_left_subsystem/1(lock/unlock)
  Front_left_passenger/1 -> Front_left_subsystem/2(In_fl_b)
  rear_left_passenger/1 -> rear_left_Subsystem/2(In2)
  rear_left_driver/1 -> rear_left_Subsystem/3(In3)
  [Lock_button2] -> rear_left_Subsystem/1(lock/unlock)
  rear_right_driver/1 -> Rear_right_Subsystem/3(rear_right_driver)
  rear_right_passenger/1 -> Rear_right_Subsystem/2(rear_right_passenger)
  [Lock_button3] -> Rear_right_Subsystem/1(lock/unlock)
  driver_side/1 -> driver_control_Subsystem/1(In1)
  Ig_sw/1 -> driver_control_Subsystem/Enable, Rear_right_Subsystem/Enable, rear_left_Subsystem/Enable, Front_left_subsystem/Enable
  object_res/1 -> Front_left_subsystem/4(object)
  Right_left_object_detc/1 -> rear_left_Subsystem/4(object)
  Obj_det_right/1 -> Rear_right_Subsystem/4(object)
  Obj_Detc_driver-side/1 -> driver_control_Subsystem/2(object)
  BCM_Door_system/1(Out1) -> Delay/1, Display/1
  DC_Acc/1 -> BCM_Door_system/1(DC_Acc)  "DC_Acc"
  DC_iginition/1 -> BCM_Door_system/2(DC_iginition)
  DC_Door1/1 -> BCM_Door_system/3(DC_Door1)
  DC_Door2/1 -> BCM_Door_system/4(DC_Door2)
  DC_Door3/1 -> BCM_Door_system/5(DC_Door3)
  DC_Door4/1 -> BCM_Door_system/6(DC_Door4)
  DC_Antilock/1 -> BCM_Door_system/7(DC_Antilock)
  BCM_Door_system/2(Out2) -> Display1/1
  BCM_Door_system/3(y) -> y/1
  BCM_Door_system/4(Outport) -> Outport/1

== system Automotive_model2/BCM_SAFETY_MODULE/BCM_WC_CONTROL ==
  note: Wiper Enabling Control:
      |
      | Switch between front, Rear and maual mode.
      | Manual control only works for front wiper
      | When user enables front wiper, he will get 6 modes including manual input.
      | WC status is to switch on/off wiper control
      | There are 3 subsystems for rear, front and manual.
  note: Wiper Control
  note: Front_Windshield
  BCM_WC_Rear_Wiper : Inport
  BCM_WC_Status : Inport  Port=2
  BCM_WC_FR_ManualINP : Inport  Port=3
  BCM_WC_FW_Modes : Inport  Port=4
  BCM_WC_FrontS : Inport  Port=5
  BCM_WC_FR_Automodes : Subsystem
  BCM_WC_FR_manual : Subsystem
  BCM_WC_FW_ENABLE : Switch  Criteria=u2 ~= 0
  BCM_WC_FW_Statuscheck : Logic  IconShape=distinctive  AllPortsSameDT=off  OutDataTypeStr=boolean
  BCM_WC_Rear_windshield : Subsystem
  Constant : Constant  Value=7
  BW_OUT : Outport
  FA_Low : Outport  Port=2
  FA_Medium : Outport  Port=3
  FA_High : Outport  Port=4
  FA_Spray : Outport  Port=5
  FA_Mist : Outport  Port=6
  FA_OFF : Outport  Port=7
  Manual_out : Outport  Port=8
  FM_lessthan30 : Outport  Port=9
  FM_Bw30_60 : Outport  Port=10
  FM_Bw60_100 : Outport  Port=11
  wires:
  BCM_WC_Status/1 -> BCM_WC_FW_Statuscheck/2, BCM_WC_Rear_windshield/2(BCM_WC_StatusINP)
  BCM_WC_FrontS/1 -> BCM_WC_FW_Statuscheck/1
  BCM_WC_FW_Statuscheck/1 -> BCM_WC_FW_ENABLE/2
  BCM_WC_FW_Modes/1 -> BCM_WC_FW_ENABLE/1
  BCM_WC_FW_ENABLE/1 -> BCM_WC_FR_Automodes/1(BCM_FR_AUTOMODES), BCM_WC_FR_manual/1(BCM_FRW_Manualmode)
  BCM_WC_Rear_Wiper/1 -> BCM_WC_Rear_windshield/1(BCM_WC_RearWiperINP)
  BCM_WC_Rear_windshield/1(BW_OUT) -> BW_OUT/1
  BCM_WC_FR_ManualINP/1 -> BCM_WC_FR_manual/2(FW_MANUAL)
  BCM_WC_FR_manual/1(BCM_FRM_Out) -> Manual_out/1
  BCM_WC_FR_manual/2(BCM_FRM_OUT1) -> FM_lessthan30/1
  BCM_WC_FR_manual/3(BCM_FRM_Bw30_60) -> FM_Bw30_60/1
  BCM_WC_FR_manual/4(BCM_FRM__Bw60_100) -> FM_Bw60_100/1
  BCM_WC_FR_Automodes/1(BCM_FR_AUTOMODE_LOWout) -> FA_Low/1
  BCM_WC_FR_Automodes/2(BCM_FR_AUTOMODE_OFF) -> FA_OFF/1
  BCM_WC_FR_Automodes/3(BCM_FR_AUTOMODE_Mediumout) -> FA_Medium/1
  BCM_WC_FR_Automodes/4(BCM_FR_AUTOMODE_High) -> FA_High/1
  BCM_WC_FR_Automodes/5(BCM_FR_AUTOMODE_Spray) -> FA_Spray/1
  BCM_WC_FR_Automodes/6(BCM_FR_AUTOMODE_Mist) -> FA_Mist/1
  Constant/1 -> BCM_WC_FW_ENABLE/3

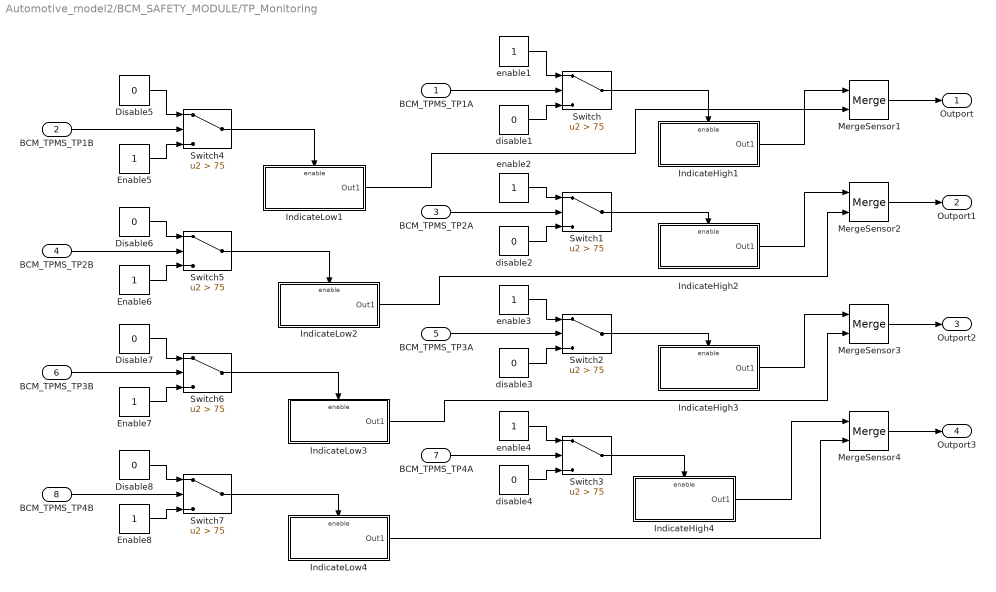
== system Automotive_model2/BCM_SAFETY_MODULE/TP_Monitoring ==
  BCM_TPMS_TP1A : Inport
  BCM_TPMS_TP1B : Inport  Port=2
  BCM_TPMS_TP2A : Inport  Port=3
  BCM_TPMS_TP2B : Inport  Port=4
  BCM_TPMS_TP3A : Inport  Port=5
  BCM_TPMS_TP3B : Inport  Port=6
  BCM_TPMS_TP4A : Inport  Port=7
  BCM_TPMS_TP4B : Inport  Port=8
  Disable{5..8} (4 alike) : Constant  Value=0
  Enable{5..8} (4 alike) : Constant
  IndicateHigh1 : Subsystem  TreatAsAtomicUnit=on
  IndicateHigh2 : Subsystem  TreatAsAtomicUnit=on
  IndicateHigh3 : Subsystem  TreatAsAtomicUnit=on
  IndicateHigh4 : Subsystem  TreatAsAtomicUnit=on
  IndicateLow1 : Subsystem  TreatAsAtomicUnit=on
  IndicateLow2 : Subsystem  TreatAsAtomicUnit=on
  IndicateLow3 : Subsystem  TreatAsAtomicUnit=on
  IndicateLow4 : Subsystem  TreatAsAtomicUnit=on
  MergeSensor{1..4} (4 alike) : Merge
  Switch{,1..7} (8 alike) : Switch  Criteria=u2 > Threshold  Threshold=75
  disable{1..4} (4 alike) : Constant  Value=0
  enable{1..4} (4 alike) : Constant
  Outport : Outport
  Outport1 : Outport  Port=2
  Outport2 : Outport  Port=3
  Outport3 : Outport  Port=4
  wires:
  enable1/1 -> Switch/1
  BCM_TPMS_TP3A/1 -> Switch2/2
  disable1/1 -> Switch/3
  disable3/1 -> Switch2/3
  enable2/1 -> Switch1/1
  BCM_TPMS_TP1A/1 -> Switch/2
  disable4/1 -> Switch3/3
  disable2/1 -> Switch1/3
  enable4/1 -> Switch3/1
  BCM_TPMS_TP2A/1 -> Switch1/2
  BCM_TPMS_TP4A/1 -> Switch3/2
  enable3/1 -> Switch2/1
  Disable8/1 -> Switch7/1
  Enable8/1 -> Switch7/3
  Disable6/1 -> Switch5/1
  Enable6/1 -> Switch5/3
  Enable7/1 -> Switch6/3
  Enable5/1 -> Switch4/3
  Disable5/1 -> Switch4/1
  BCM_TPMS_TP2B/1 -> Switch5/2
  BCM_TPMS_TP3B/1 -> Switch6/2
  BCM_TPMS_TP1B/1 -> Switch4/2
  Disable7/1 -> Switch6/1
  BCM_TPMS_TP4B/1 -> Switch7/2
  Switch3/1 -> IndicateHigh4/Enable
  Switch2/1 -> IndicateHigh3/Enable
  Switch1/1 -> IndicateHigh2/Enable
  Switch/1 -> IndicateHigh1/Enable
  Switch7/1 -> IndicateLow4/Enable
  Switch6/1 -> IndicateLow3/Enable
  Switch5/1 -> IndicateLow2/Enable
  Switch4/1 -> IndicateLow1/Enable
  IndicateHigh1/1(Out1) -> MergeSensor1/1
  IndicateLow1/1(Out1) -> MergeSensor1/2
  IndicateHigh2/1(Out1) -> MergeSensor2/1
  IndicateLow2/1(Out1) -> MergeSensor2/2
  IndicateHigh3/1(Out1) -> MergeSensor3/1
  IndicateLow3/1(Out1) -> MergeSensor3/2
  IndicateHigh4/1(Out1) -> MergeSensor4/1
  IndicateLow4/1(Out1) -> MergeSensor4/2
  MergeSensor1/1 -> Outport/1
  MergeSensor2/1 -> Outport1/1
  MergeSensor3/1 -> Outport2/1
  MergeSensor4/1 -> Outport3/1

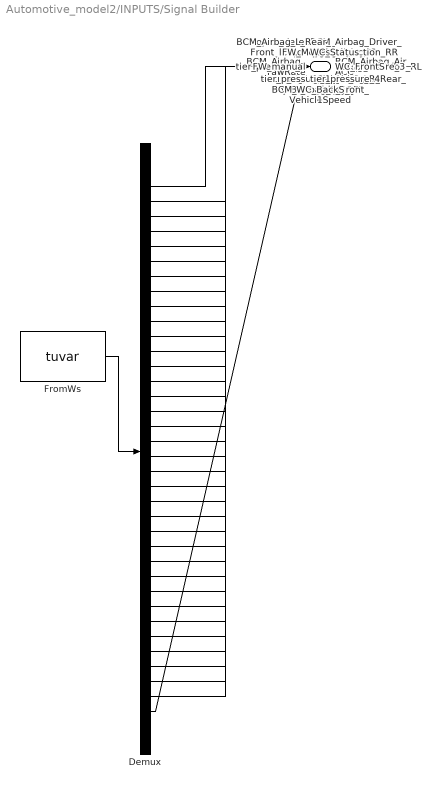
== system Automotive_model2/INPUTS/Signal Builder ==
  Demux : Demux  Tag=STV Demux  Outputs=36
      settings: DisplayOption=none
  FromWs : FromWorkspace  Tag=STV FromWs  VariableName=tuvar
      SigBuilderData=|
      | common.afterFinalStr = 'Extrapolate'
      | common.sampleTime = '0'
      | dataSet.timeRange = [0 97]
      | dataSet.name = 'Sheet1'
      | sbobj.Name = 'Signal Builder'
      | sbobj.Groups.Name = 'Sheet1'
      | sbobj.Groups.Signals(1).Name = 'Front_left_CP'
      | sbobj.Groups.Signals(1).XData = [0 1 2 3 4 5 6 7 8 9 10 11 12 13 14 15 16 17 18 19 20 21 22 23 24 25 26 27 28 29 30 31 32 33 34 35 36 37 38 39 40 41 42 43 44 45 46 47 48 49 50 51 52 53 54 55 56 57 58 59 60 61 62 63 64 65 66 67 68 69 70 71 72 73 74 75 76 77 78 79 80 81 82 83 84 85 86 87 88 89 90 91 92 93 94 95 96 97]
      | sbobj.Groups.Signals(1).YData = [0 0 0 0 0 0 0 1 1 1 1 1 1 1 1 -1 -1 -1 -1 -1 0 1 1 0 -1 -1 1 1 1 0 0 1 1 1 1 0 -1 -1 -1 -1 0 1 1 -1 -1 1 1 1 0 0 0 0 0 0 0 0 1 1 1 1 1 0 0 1 0 0 0 0 0 0 0 0 0 0 0 0 1 1 1 1 -1 -1 1 1 1 0 0 0 0 0 0 0 0 0 0 0 0 0]
      | sbobj.Groups.Signals(2).Name = 'Right_left_CP'
      | sbobj.Groups.Signals(2).XData = [0 1 2 3 4 5 6 7 8 9 10 11 12 13 14 15 16 17 18 19 20 21 22 23 24 25 26 27 28 29 30 31 32 33 34 35 36 37 38 39 40 41 42 43 44 45 46 47 48 49 50 51 52 53 54 55 56 57 58 59 60 61 62 63 64 65 66 67 68 69 70 71 72 73 74 75 76 77 78 79 80 81 82 83 84 85 86 87 88 89 90 91 92 93 94 95 96 97]
      | sbobj.Groups.Signals(2).YData = [0 0 0 0 0 0 0 1 1 1 1 1 1 1 1 -1 -1 -1 -1 -1 0 1 1 0 -1 -1 1 1 1 0 0 1 1 1 1 0 -1 -1 -1 -1 0 1 1 -1 -1 1 1 1 0 0 0 0 0 0 0 0 1 1 1 1 1 0 0 1 0 0 0 0 0 0 0 0 0 0 0 0 1 1 1 1 -1 -1 1 1 1 0 0 0 0 0 0 0 0 0 0 0 0 0]
      | sbobj.Groups.Signals(3).Name = 'Right_right_CP'
      | sbobj.Groups.Signals(3).XData = [0 1 2 3 4 5 6 7 8 9 10 11 12 13 14 15 16 17 18 19 20 21 22 23 24 25 26 27 28 29 30 31 32 33 34 35 36 37 38 39 40 41 42 43 44 45 46 47 48 49 50 51 52 53 54 55 56 57 58 59 60 61 62 63 64 65 66 67 68 69 70 71 72 73 74 75 76 77 78 79 80 81 82 83 84 85 86 87 88 89 90 91 92 93 94 95 96 97]
      | sbobj.Groups.Signals(3).YData = [1 1 0 0 -1 -1 0 1 1 1 1 1 1 1 1 -1 -1 -1 -1 -1 0 1 1 0 -1 -1 1 1 1 0 0 1 1 1 1 0 -1 -1 -1 -1 0 1 1 -1 -1 1 1 1 0 0 0 0 0 0 0 0 1 1 1 1 1 0 0 1 0 0 0 0 0 0 0 0 0 0 0 0 1 1 1 1 -1 -1 1 1 1 0 0 0 0 0 0 0 0 0 0 0 0 0]
      | sbobj.Groups.Signals(4).Name = 'Driver_control'
      | sbobj.Groups.Signals(4).XData = [0 1 2 3 4 5 6 7 8 9 10 11 12 13 14 15 16 17 18 19 20 21 22 23 24 25 26 27 28 29 30 31 32 33 34 35 36 37 38 39 40 41 42 43 44 45 46 47 48 49 50 51 52 53 54 55 56 57 58 59 60 61 62 63 64 65 66 67 68 69 70 71 72 73 74 75 76 77 78 79 80 81 82 83 84 85 86 87 88 89 90 91 92 93 94 95 96 97]
      | sbobj.Groups.Signals(4).YData = [0 0 0 0 0 0 0 1 1 1 1 1 1 1 1 -1 -1 -1 -1 -1 0 1 1 0 -1 -1 1 1 1 1 1 1 1 1 -1 -1 -1 -1 0 1 1 -1 -1 1 1 1 1 1 0 0 0 0 0 0 0 0 1 1 1 1 1 0 0 1 0 0 0 0 0 0 0 0 0 0 0 0 1 1 1 -1 1 1 1 1 1 0 0 0 0 0 0 0 0 0 0 0 0 0]
      | sbobj.Groups.Signals(5).Name = 'Front_left_DC'
      | sbobj.Groups.Signals(5).XData = [0 1 2 3 4 5 6 7 8 9 10 11 12 13 14 15 16 17 18 19 20 21 22 23 24 25 26 27 28 29 30 31 32 33 34 35 36 37 38 39 40 41 42 43 44 45 46 47 48 49 50 51 52 53 54 55 56 57 58 59 60 61 62 63 64 65 66 67 68 69 70 71 72 73 74 75 76 77 78 79 80 81 82 83 84 85 86 87 88 89 90 91 92 93 94 95 96 97]
      | sbobj.Groups.Signals(5).YData = [0 0 0 -1 1 0 0 1 1 1 1 1 1 1 0 -1 -1 -1 -1 -1 0 1 1 0 -1 -1 1 1 1 1 1 -1 0 1 0 0 0 0 0 0 0 0 0 0 0 1 1 1 0 0 0 0 0 0 0 0 1 1 1 1 1 0 0 1 0 0 0 0 0 0 0 0 0 0 0 0 1 1 1 0 0 0 1 1 1 0 0 0 0 0 0 0 0 0 0 0 0 0]
      | sbobj.Groups.Signals(6).Name = 'rear_left_DC'
      | sbobj.Groups.Signals(6).XData = [0 1 2 3 4 5 6 7 8 9 10 11 12 13 14 15 16 17 18 19 20 21 22 23 24 25 26 27 28 29 30 31 32 33 34 35 36 37 38 39 40 41 42 43 44 45 46 47 48 49 50 51 52 53 54 55 56 57 58 59 60 61 62 63 64 65 66 67 68 69 70 71 72 73 74 75 76 77 78 79 80 81 82 83 84 85 86 87 88 89 90 91 92 93 94 95 96 97]
      | sbobj.Groups.Signals(6).YData = [0 0 0 0 0 0 0 1 1 1 1 1 1 1 1 -1 -1 -1 -1 -1 0 1 1 0 -1 -1 1 1 1 1 1 0 -1 1 0 0 0 0 0 0 0 0 0 0 0 1 1 1 0 0 0 0 0 0 0 0 1 1 1 1 1 0 0 1 0 0 0 0 0 0 0 0 0 0 0 0 1 1 1 0 0 0 1 1 1 0 0 0 0 0 0 0 0 0 0 0 0 0]
      | sbobj.Groups.Signals(7).Name = 'rear_right_DC'
      | sbobj.Groups.Signals(7).XData = [0 1 2 3 4 5 6 7 8 9 10 11 12 13 14 15 16 17 18 19 20 21 22 23 24 25 26 27 28 29 30 31 32 33 34 35 36 37 38 39 40 41 42 43 44 45 46 47 48 49 50 51 52 53 54 55 56 57 58 59 60 61 62 63 64 65 66 67 68 69 70 71 72 73 74 75 76 77 78 79 80 81 82 83 84 85 86 87 88 89 90 91 92 93 94 95 96 97]
      | sbobj.Groups.Signals(7).YData = [0 0 0 0 0 0 0 1 1 1 1 1 1 1 1 -1 -1 -1 -1 -1 0 1 1 0 -1 -1 1 -1 0 1 1 0 0 1 0 0 0 0 0 0 0 0 0 0 0 1 1 1 0 0 0 0 0 0 0 0 1 1 1 1 1 0 0 1 0 0 0 0 0 0 0 0 0 0 0 0 1 1 1 0 0 0 1 1 1 0 0 0 0 0 0 0 0 0 0 0 0 0]
      | sbobj.Groups.Signals(8).Name = 'oject_detection_FL'
      | sbobj.Groups.Signals(8).XData = [0 1 2 3 4 5 6 7 8 9 10 11 12 13 14 15 16 17 18 19 20 21 22 23 24 25 26 27 28 29 30 31 32 33 34 35 36 37 38 39 40 41 42 43 44 45 46 47 48 49 50 51 52 53 54 55 56 57 58 59 60 61 62 63 64 65 66 67 68 69 70 71 72 73 74 75 76 77 78 79 80 81 82 83 84 85 86 87 88 89 90 91 92 93 94 95 96 97]
      | sbobj.Groups.Signals(8).YData = [1 1 1 0 0 1 0 0 0 0 0 0 0 1 1 0 0 0 0 1 0 0 0 0 0 1 1 1 1 1 0 0 1 1 0 0 0 0 0 0 0 0 0 0 0 1 1 1 0 0 0 0 0 0 0 0 1 1 1 1 1 0 0 1 0 0 0 0 0 0 0 0 0 0 0 0 1 1 1 0 0 0 1 1 1 0 0 0 0 0 0 0 0 0 0 0 0 0]
      | sbobj.Groups.Signals(9).Name = 'Lock_Unlock'
      | sbobj.Groups.Signals(9).XData = [0 1 2 3 4 5 6 7 8 9 10 11 12 13 14 15 16 17 18 19 20 21 22 23 24 25 26 27 28 29 30 31 32 33 34 35 36 37 38 39 40 41 42 43 44 45 46 47 48 49 50 51 52 53 54 55 56 57 58 59 60 61 62 63 64 65 66 67 68 69 70 71 72 73 74 75 76 77 78 79 80 81 82 83 84 85 86 87 88 89 90 91 92 93 94 95 96 97]
      | sbobj.Groups.Signals(9).YData = [1 0 1 0 1 0 0 0 0 0 0 0 0 0 0 0 0 0 0 0 0 0 0 0 0 0 0 0 0 1 1 1 1 1 1 1 1 1 1 1 1 1 1 1 1 1 1 1 0 0 0 0 0 0 0 0 1 1 1 1 1 0 0 1 0 0 0 0 0 0 0 0 0 0 0 0 1 1 1 1 1 1 1 1 1 0 0 0 0 0 0 0 0 0 0 0 0 0]
      | sbobj.Groups.Signals(10).Name = 'iginition'
      | sbobj.Groups.Signals(10).XData = [0 1 2 3 4 5 6 7 8 9 10 11 12 13 14 15 16 17 18 19 20 21 22 23 24 25 26 27 28 29 30 31 32 33 34 35 36 37 38 39 40 41 42 43 44 45 46 47 48 49 50 51 52 53 54 55 56 57 58 59 60 61 62 63 64 65 66 67 68 69 70 71 72 73 74 75 76 77 78 79 80 81 82 83 84 85 86 87 88 89 90 91 92 93 94 95 96 97]
      | sbobj.Groups.Signals(10).YData = [0 0 0 0 0 0 0 1 1 1 1 1 1 1 1 1 1 1 1 1 1 1 1 1 1 1 1 1 1 1 1 1 1 1 1 1 1 1 1 1 1 1 1 1 1 1 1 1 0 0 0 0 0 0 0 0 1 1 1 1 1 0 0 1 0 0 0 0 0 0 0 0 0 0 0 0 1 1 1 1 1 1 1 1 1 0 0 0 0 0 0 0 0 0 0 0 0 0]
      | sbobj.Groups.Signals(11).Name = 'oject_detection_RL'
      | sbobj.Groups.Signals(11).XData = [0 1 2 3 4 5 6 7 8 9 10 11 12 13 14 15 16 17 18 19 20 21 22 23 24 25 26 27 28 29 30 31 32 33 34 35 36 37 38 39 40 41 42 43 44 45 46 47 48 49 50 51 52 53 54 55 56 57 58 59 60 61 62 63 64 65 66 67 68 69 70 71 72 73 74 75 76 77 78 79 80 81 82 83 84 85 86 87 88 89 90 91 92 93 94 95 96 97]
      | sbobj.Groups.Signals(11).YData = [1 1 1 0 0 1 0 0 0 0 0 0 0 1 1 0 0 0 0 1 0 0 0 0 0 1 1 1 1 1 0 0 1 0 1 1 0 0 0 0 0 0 0 0 0 1 1 1 0 0 0 0 0 0 0 0 1 1 1 1 1 0 0 1 0 0 0 0 0 0 0 0 0 0 0 0 1 1 1 0 0 0 1 1 1 0 0 0 0 0 0 0 0 0 0 0 0 0]
      | sbobj.Groups.Signals(12).Name = 'oject_detection_RR'
      | sbobj.Groups.Signals(12).XData = [0 1 2 3 4 5 6 7 8 9 10 11 12 13 14 15 16 17 18 19 20 21 22 23 24 25 26 27 28 29 30 31 32 33 34 35 36 37 38 39 40 41 42 43 44 45 46 47 48 49 50 51 52 53 54 55 56 57 58 59 60 61 62 63 64 65 66 67 68 69 70 71 72 73 74 75 76 77 78 79 80 81 82 83 84 85 86 87 88 89 90 91 92 93 94 95 96 97]
      | sbobj.Groups.Signals(12).YData = [1 1 1 0 0 1 0 0 0 0 0 0 0 1 1 0 0 0 0 1 0 0 0 0 0 1 1 1 1 1 0 0 1 0 1 1 0 0 0 0 0 0 0 0 0 1 1 1 0 0 0 0 0 0 0 0 1 1 1 1 1 0 0 1 0 0 0 0 0 0 0 0 0 0 0 0 1 1 1 0 0 0 1 1 1 0 0 0 0 0 0 0 0 0 0 0 0 0]
      | sbobj.Groups.Signals(13).Name = 'oject_detection_driver'
      | sbobj.Groups.Signals(13).XData = [0 1 2 3 4 5 6 7 8 9 10 11 12 13 14 15 16 17 18 19 20 21 22 23 24 25 26 27 28 29 30 31 32 33 34 35 36 37 38 39 40 41 42 43 44 45 46 47 48 49 50 51 52 53 54 55 56 57 58 59 60 61 62 63 64 65 66 67 68 69 70 71 72 73 74 75 76 77 78 79 80 81 82 83 84 85 86 87 88 89 90 91 92 93 94 95 96 97]
      | sbobj.Groups.Signals(13).YData = [1 1 1 0 0 1 0 0 0 0 0 0 0 1 0 0 0 0 0 1 0 0 0 0 0 1 1 1 1 1 0 0 1 0 1 1 0 0 0 0 0 0 0 0 0 1 1 1 0 0 0 0 0 0 0 0 1 1 1 1 1 0 0 1 0 0 0 0 0 0 0 0 0 0 0 0 1 1 1 0 0 0 1 1 1 0 0 0 0 0 0 0 0 0 0 0 0 0]
      | sbobj.Groups.Signals(14).Name = 'ignition status'
      | sbobj.Groups.Signals(14).XData = [0 1 2 3 4 5 6 7 8 9 10 11 12 13 14 15 16 17 18 19 20 21 22 23 24 25 26 27 28 29 30 31 32 33 34 35 36 37 38 39 40 41 42 43 44 45 46 47 48 49 50 51 52 53 54 55 56 57 58 59 60 61 62 63 64 65 66 67 68 69 70 71 72 73 74 75 76 77 78 79 80 81 82 83 84 85 86 87 88 89 90 91 92 93 94 95 96 97]
      | sbobj.Groups.Signals(14).YData = [1 1 1 1 1 1 0 0 0 0 0 0 1 1 1 1 1 1 1 1 1 1 0 0 0 0 0 0 0 0 0 0 0 0 0 0 0 0 0 0 0 0 1 1 1 1 1 1 1 1 0 0 0 0 0 0 0 0 0 0 0 0 0 0 1 1 1 1 0 0 0 0 0 0 0 0 0 0 0 1 1 1 1 1 1 1 1 0 0 0 0 0 0 0 0 0 0 0]
      | sbobj.Groups.Signals(15).Name = 'Door_1'
      | sbobj.Groups.Signals(15).XData = [0 1 2 3 4 5 6 7 8 9 10 11 12 13 14 15 16 17 18 19 20 21 22 23 24 25 26 27 28 29 30 31 32 33 34 35 36 37 38 39 40 41 42 43 44 45 46 47 48 49 50 51 52 53 54 55 56 57 58 59 60 61 62 63 64 65 66 67 68 69 70 71 72 73 74 75 76 77 78 79 80 81 82 83 84 85 86 87 88 89 90 91 92 93 94 95 96 97]
      | sbobj.Groups.Signals(15).YData = [1 1 1 1 1 1 1 1 1 1 1 1 1 1 1 1 1 1 1 1 1 1 0 0 0 0 0 0 0 1 1 1 1 1 1 1 1 1 1 1 1 1 1 1 1 1 1 1 1 0 0 0 0 0 0 0 0 0 0 0 0 0 0 0 0 0 0 0 0 0 0 0 0 0 0 0 0 0 0 1 1 1 1 1 1 1 0 0 0 0 0 0 0 0 0 0 0 0]
      | sbobj.Groups.Signals(16).Name = 'Door_2'
      | sbobj.Groups.Signals(16).XData = [0 1 2 3 4 5 6 7 8 9 10 11 12 13 14 15 16 17 18 19 20 21 22 23 24 25 26 27 28 29 30 31 32 33 34 35 36 37 38 39 40 41 42 43 44 45 46 47 48 49 50 51 52 53 54 55 56 57 58 59 60 61 62 63 64 65 66 67 68 69 70 71 72 73 74 75 76 77 78 79 80 81 82 83 84 85 86 87 88 89 90 91 92 93 94 95 96 97]
      | sbobj.Groups.Signals(16).YData = [1 1 1 1 1 1 1 1 1 1 1 1 1 1 1 1 1 1 1 1 1 1 0 0 0 0 0 0 0 0 0 0 0 0 0 0 0 0 0 0 0 0 0 0 0 0 0 0 0 0 0 0 0 0 0 0 0 0 0 0 0 1 1 1 1 1 1 1 1 1 1 1 1 1 1 1 1 1 1 1 1 1 1 1 1 1 1 1 1 1 1 0 0 0 0 0 0 0]
      | sbobj.Groups.Signals(17).Name = 'Door_3'
      | sbobj.Groups.Signals(17).XData = [0 1 2 3 4 5 6 7 8 9 10 11 12 13 14 15 16 17 18 19 20 21 22 23 24 25 26 27 28 29 30 31 32 33 34 35 36 37 38 39 40 41 42 43 44 45 46 47 48 49 50 51 52 53 54 55 56 57 58 59 60 61 62 63 64 65 66 67 68 69 70 71 72 73 74 75 76 77 78 79 80 81 82 83 84 85 86 87 88 89 90 91 92 93 94 95 96 97]
      | sbobj.Groups.Signals(17).YData = [1 1 1 1 1 1 1 1 1 1 1 1 1 1 1 1 1 1 1 1 1 1 0 0 0 0 0 0 0 1 1 1 1 1 1 1 1 1 1 1 1 0 0 0 0 0 0 0 0 0 0 1 1 1 1 0 0 0 0 0 0 0 0 0 0 0 0 0 0 1 1 1 1 1 1 1 1 1 1 1 1 1 1 1 1 1 1 1 1 1 1 0 0 0 0 0 0 0]
      | sbobj.Groups.Signals(18).Name = 'Door_4'
      | sbobj.Groups.Signals(18).XData = [0 1 2 3 4 5 6 7 8 9 10 11 12 13 14 15 16 17 18 19 20 21 22 23 24 25 26 27 28 29 30 31 32 33 34 35 36 37 38 39 40 41 42 43 44 45 46 47 48 49 50 51 52 53 54 55 56 57 58 59 60 61 62 63 64 65 66 67 68 69 70 71 72 73 74 75 76 77 78 79 80 81 82 83 84 85 86 87 88 89 90 91 92 93 94 95 96 97]
      | sbobj.Groups.Signals(18).YData = [1 1 1 1 1 1 1 1 1 1 1 1 1 1 1 1 1 1 1 1 1 1 0 0 0 0 0 0 0 1 1 1 1 1 1 1 1 1 1 1 1 1 1 1 1 1 1 1 1 1 1 0 0 0 0 0 0 0 0 0 0 0 0 0 0 0 0 0 0 0 0 0 0 0 0 0 0 0 0 0 0 0 0 0 0 0 0 0 0 0 1 1 1 1 1 1 1 1]
      | sbobj.Groups.Signals(19).Name = 'antilockleature'
      | sbobj.Groups.Signals(19).XData = [0 1 2 3 4 5 6 7 8 9 10 11 12 13 14 15 16 17 18 19 20 21 22 23 24 25 26 27 28 29 30 31 32 33 34 35 36 37 38 39 40 41 42 43 44 45 46 47 48 49 50 51 52 53 54 55 56 57 58 59 60 61 62 63 64 65 66 67 68 69 70 71 72 73 74 75 76 77 78 79 80 81 82 83 84 85 86 87 88 89 90 91 92 93 94 95 96 97]
      | sbobj.Groups.Signals(19).YData = [1 1 1 1 1 1 1 1 1 1 1 1 1 1 1 1 1 1 1 1 1 1 1 1 0 0 0 0 0 1 1 1 1 1 1 1 1 1 1 1 1 1 1 1 1 1 1 1 1 1 1 0 0 0 0 0 0 0 1 1 1 1 1 1 1 1 1 1 1 1 1 1 1 1 1 1 1 1 0 0 0 0 0 0 0 0 0 0 0 0 0 0 0 0 0 0 0 1]
      | sbobj.Groups.Signals(20).Name = 'accln'
      | sbobj.Groups.Signals(20).XData = [0 1 2 3 4 5 6 7 8 9 10 11 12 13 14 15 16 17 18 19 20 21 22 23 24 25 26 27 28 29 30 31 32 33 34 35 36 37 38 39 40 41 42 43 44 45 46 47 48 49 50 51 52 53 54 55 56 57 58 59 60 61 62 63 64 65 66 67 68 69 70 71 72 73 74 75 76 77 78 79 80 81 82 83 84 85 86 87 88 89 90 91 92 93 94 95 96 97]
      | sbobj.Groups.Signals(20).YData = [13 14 15 16 17 18 12 20 21 9 10 25 27 29 31 33 35 37 39 41 43 45 47 49 51 53 55 57 59 1 4 5 6 7 8 9 10 11 12 2 3 4 5 6 7 8 9 10 11 21 22 23 24 25 26 27 28 29 30 31 32 1 2 3 4 5 6 7 8 9 10 11 20 21 22 23 24 25 26 27 28 29 30 31 32 33 34 35 36 37 38 39 40 41 42 9 10 11]
      | sbobj.Groups.Signals(21).Name = 'BCM_Airbag_VehicleSpeed'
      | sbobj.Groups.Signals(21).XData = [0 1 2 3 4 5 6 7 8 9 10 11 12 13 14 15 16 17 18 19 20 21 22 23 24 25 26 27 28 29 30 31 32 33 34 35 36 37 38 39 40 41 42 43 44 45 46 47 48 49 50 51 52 53 54 55 56 57 58 59 60 61 62 63 64 65 66 67 68 69 70 71 72 73 74 75 76 77 78 79 80 81 82 83 84 85 86 87 88 89 90 91 92 93 94 95 96 97]
      | sbobj.Groups.Signals(21).YData = [50 50 140 140 140 140 140 140 140 140 140 140 140 140 140 140 140 140 140 140 140 140 140 140 140 140 140 140 140 140 140 140 140 0 0 0 0 0 0 0 0 0 0 0 0 0 0 0 0 0 0 0 0 0 0 0 0 0 0 0 0 0 0 0 0 0 0 0 0 0 0 0 0 0 0 0 0 0 0 0 0 0 0 0 0 0 0 0 0 0 0 0 0 0 0 0 0 0]
      | sbobj.Groups.Signals(22).Name = 'BCM_Airbag_YawRate'
      | sbobj.Groups.Signals(22).XData = [0 1 2 3 4 5 6 7 8 9 10 11 12 13 14 15 16 17 18 19 20 21 22 23 24 25 26 27 28 29 30 31 32 33 34 35 36 37 38 39 40 41 42 43 44 45 46 47 48 49 50 51 52 53 54 55 56 57 58 59 60 61 62 63 64 65 66 67 68 69 70 71 72 73 74 75 76 77 78 79 80 81 82 83 84 85 86 87 88 89 90 91 92 93 94 95 96 97]
      | sbobj.Groups.Signals(22).YData = [50 100 100 100 100 100 100 100 100 100 100 100 100 100 100 100 100 100 50 50 50 50 50 50 50 50 50 50 50 50 50 50 50 0 100 50 100 50 0 0 0 0 0 0 0 0 0 0 0 0 0 0 0 0 0 0 0 0 0 0 0 0 0 0 0 0 0 0 0 0 0 0 0 0 0 0 0 0 0 0 0 0 0 0 0 0 0 0 0 0 0 0 0 0 0 0 0 0]
      | sbobj.Groups.Signals(23).Name = 'BCM_Airbag_Air_ACC'
      | sbobj.Groups.Signals(23).XData = [0 1 2 3 4 5 6 7 8 9 10 11 12 13 14 15 16 17 18 19 20 21 22 23 24 25 26 27 28 29 30 31 32 33 34 35 36 37 38 39 40 41 42 43 44 45 46 47 48 49 50 51 52 53 54 55 56 57 58 59 60 61 62 63 64 65 66 67 68 69 70 71 72 73 74 75 76 77 78 79 80 81 82 83 84 85 86 87 88 89 90 91 92 93 94 95 96 97]
      | sbobj.Groups.Signals(23).YData = [0 0 1 1 1 1 1 1 1 1 1 1 1 1 1 1 1 1 1 1 1 1 1 1 1 1 1 1 1 1 1 1 1 0 0 0 0 0 0 0 0 0 0 0 0 0 0 0 0 0 0 0 0 0 0 0 0 0 0 0 0 0 0 0 0 0 0 0 0 0 0 0 0 0 0 0 0 0 0 0 0 0 0 0 0 0 0 0 0 0 0 0 0 0 0 0 0 0]
      | sbobj.Groups.Signals(24).Name = 'BCM_Airbag_Driver_L'
      | sbobj.Groups.Signals(24).XData = [0 1 2 3 4 5 6 7 8 9 10 11 12 13 14 15 16 17 18 19 20 21 22 23 24 25 26 27 28 29 30 31 32 33 34 35 36 37 38 39 40 41 42 43 44 45 46 47 48 49 50 51 52 53 54 55 56 57 58 59 60 61 62 63 64 65 66 67 68 69 70 71 72 73 74 75 76 77 78 79 80 81 82 83 84 85 86 87 88 89 90 91 92 93 94 95 96 97]
      | sbobj.Groups.Signals(24).YData = [0 0 0 0 0 0 0 0 0 0 1 1 1 1 1 1 1 1 0 0 0 0 0 0 0 1 1 1 1 1 1 1 1 0 0 0 0 0 0 0 0 0 0 0 0 0 0 0 0 0 0 0 0 0 0 0 0 0 0 0 0 0 0 0 0 0 0 0 0 0 0 0 0 0 0 0 0 0 0 0 0 0 0 0 0 0 0 0 0 0 0 0 0 0 0 0 0 0]
      | sbobj.Groups.Signals(25).Name = 'BCM_Airbag_L_Front_1'
      | sbobj.Groups.Signals(25).XData = [0 1 2 3 4 5 6 7 8 9 10 11 12 13 14 15 16 17 18 19 20 21 22 23 24 25 26 27 28 29 30 31 32 33 34 35 36 37 38 39 40 41 42 43 44 45 46 47 48 49 50 51 52 53 54 55 56 57 58 59 60 61 62 63 64 65 66 67 68 69 70 71 72 73 74 75 76 77 78 79 80 81 82 83 84 85 86 87 88 89 90 91 92 93 94 95 96 97]
      | sbobj.Groups.Signals(25).YData = [0 0 0 0 0 0 1 1 1 1 0 0 0 0 1 1 1 1 0 0 0 1 1 1 1 0 0 0 0 1 1 1 1 0 0 0 0 0 0 0 0 0 0 0 0 0 0 0 0 0 0 0 0 0 0 0 0 0 0 0 0 0 0 0 0 0 0 0 0 0 0 0 0 0 0 0 0 0 0 0 0 0 0 0 0 0 0 0 0 0 0 0 0 0 0 0 0 0]
      | sbobj.Groups.Signals(26).Name = 'BCM_Airbag_L_Rear_1'
      | sbobj.Groups.Signals(26).XData = [0 1 2 3 4 5 6 7 8 9 10 11 12 13 14 15 16 17 18 19 20 21 22 23 24 25 26 27 28 29 30 31 32 33 34 35 36 37 38 39 40 41 42 43 44 45 46 47 48 49 50 51 52 53 54 55 56 57 58 59 60 61 62 63 64 65 66 67 68 69 70 71 72 73 74 75 76 77 78 79 80 81 82 83 84 85 86 87 88 89 90 91 92 93 94 95 96 97]
      | sbobj.Groups.Signals(26).YData = [0 0 0 0 1 1 0 0 1 1 0 0 1 1 0 0 1 1 0 1 1 0 0 1 1 0 0 1 1 0 0 1 1 0 0 0 0 0 0 0 0 0 0 0 0 0 0 0 0 0 0 0 0 0 0 0 0 0 0 0 0 0 0 0 0 0 0 0 0 0 0 0 0 0 0 0 0 0 0 0 0 0 0 0 0 0 0 0 0 0 0 0 0 0 0 0 0 0]
      | sbobj.Groups.Signals(27).Name = 'BCM_Airbag_R_Rear_'
      | sbobj.Groups.Signals(27).XData = [0 1 2 3 4 5 6 7 8 9 10 11 12 13 14 15 16 17 18 19 20 21 22 23 24 25 26 27 28 29 30 31 32 33 34 35 36 37 38 39 40 41 42 43 44 45 46 47 48 49 50 51 52 53 54 55 56 57 58 59 60 61 62 63 64 65 66 67 68 69 70 71 72 73 74 75 76 77 78 79 80 81 82 83 84 85 86 87 88 89 90 91 92 93 94 95 96 97]
      | sbobj.Groups.Signals(27).YData = [0 0 0 1 0 1 0 1 0 1 0 1 0 1 0 1 0 1 1 0 1 0 1 0 1 0 1 0 1 0 1 0 1 0 0 0 0 0 0 0 0 0 0 0 0 0 0 0 0 0 0 0 0 0 0 0 0 0 0 0 0 0 0 0 0 0 0 0 0 0 0 0 0 0 0 0 0 0 0 0 0 0 0 0 0 0 0 0 0 0 0 0 0 0 0 0 0 0]
      | sbobj.Groups.Signals(28).Name = 'tier_pressure_1'
      | sbobj.Groups.Signals(28).XData = [0 1 2 3 4 5 6 7 8 9 10 11 12 13 14 15 16 17 18 19 20 21 22 23 24 25 26 27 28 29 30 31 32 33 34 35 36 37 38 39 40 41 42 43 44 45 46 47 48 49 50 51 52 53 54 55 56 57 58 59 60 61 62 63 64 65 66 67 68 69 70 71 72 73 74 75 76 77 78 79 80 81 82 83 84 85 86 87 88 89 90 91 92 93 94 95 96 97]
      | sbobj.Groups.Signals(28).YData = [88 88 88 88 88 88 88 88 88 88 88 88 88 88 88 88 88 88 88 88 55 55 55 88 55 55 55 55 55 55 55 55 0 0 0 0 0 0 0 0 0 0 0 0 0 0 0 0 0 0 0 0 0 0 0 0 0 0 0 0 0 0 0 0 0 0 0 0 0 0 0 0 0 0 0 0 0 0 0 0 0 0 0 0 0 0 0 0 0 0 0 0 0 0 0 0 0 0]
      | sbobj.Groups.Signals(29).Name = 'tier_pressure_2'
      | sbobj.Groups.Signals(29).XData = [0 1 2 3 4 5 6 7 8 9 10 11 12 13 14 15 16 17 18 19 20 21 22 23 24 25 26 27 28 29 30 31 32 33 34 35 36 37 38 39 40 41 42 43 44 45 46 47 48 49 50 51 52 53 54 55 56 57 58 59 60 61 62 63 64 65 66 67 68 69 70 71 72 73 74 75 76 77 78 79 80 81 82 83 84 85 86 87 88 89 90 91 92 93 94 95 96 97]
      | sbobj.Groups.Signals(29).YData = [88 88 88 88 55 55 55 55 88 88 88 88 88 88 88 88 55 55 55 55 88 88 88 88 88 88 88 88 55 55 55 55 0 0 0 0 0 0 0 0 0 0 0 0 0 0 0 0 0 0 0 0 0 0 0 0 0 0 0 0 0 0 0 0 0 0 0 0 0 0 0 0 0 0 0 0 0 0 0 0 0 0 0 0 0 0 0 0 0 0 0 0 0 0 0 0 0 0]
      | sbobj.Groups.Signals(30).Name = 'tier_pressure_3'
      | sbobj.Groups.Signals(30).XData = [0 1 2 3 4 5 6 7 8 9 10 11 12 13 14 15 16 17 18 19 20 21 22 23 24 25 26 27 28 29 30 31 32 33 34 35 36 37 38 39 40 41 42 43 44 45 46 47 48 49 50 51 52 53 54 55 56 57 58 59 60 61 62 63 64 65 66 67 68 69 70 71 72 73 74 75 76 77 78 79 80 81 82 83 84 85 86 87 88 89 90 91 92 93 94 95 96 97]
      | sbobj.Groups.Signals(30).YData = [88 88 55 55 88 88 55 55 88 88 55 55 88 88 55 55 88 88 55 55 88 88 55 55 88 88 55 55 88 88 55 55 0 0 0 0 0 0 0 0 0 0 0 0 0 0 0 0 0 0 0 0 0 0 0 0 0 0 0 0 0 0 0 0 0 0 0 0 0 0 0 0 0 0 0 0 0 0 0 0 0 0 0 0 0 0 0 0 0 0 0 0 0 0 0 0 0 0]
      | sbobj.Groups.Signals(31).Name = 'tier_pressure_4'
      | sbobj.Groups.Signals(31).XData = [0 1 2 3 4 5 6 7 8 9 10 11 12 13 14 15 16 17 18 19 20 21 22 23 24 25 26 27 28 29 30 31 32 33 34 35 36 37 38 39 40 41 42 43 44 45 46 47 48 49 50 51 52 53 54 55 56 57 58 59 60 61 62 63 64 65 66 67 68 69 70 71 72 73 74 75 76 77 78 79 80 81 82 83 84 85 86 87 88 89 90 91 92 93 94 95 96 97]
      | sbobj.Groups.Signals(31).YData = [88 55 88 55 88 55 88 55 88 55 88 55 88 55 88 55 88 55 88 55 88 55 88 55 88 55 88 55 88 55 88 55 0 0 0 0 0 0 0 0 0 0 0 0 0 0 0 0 0 0 0 0 0 0 0 0 0 0 0 0 0 0 0 0 0 0 0 0 0 0 0 0 0 0 0 0 0 0 0 0 0 0 0 0 0 0 0 0 0 0 0 0 0 0 0 0 0 0]
      | sbobj.Groups.Signals(32).Name = 'FW_Modes'
      | sbobj.Groups.Signals(32).XData = [0 1 2 3 4 5 6 7 8 9 10 11 12 13 14 15 16 17 18 19 20 21 22 23 24 25 26 27 28 29 30 31 32 33 34 35 36 37 38 39 40 41 42 43 44 45 46 47 48 49 50 51 52 53 54 55 56 57 58 59 60 61 62 63 64 65 66 67 68 69 70 71 72 73 74 75 76 77 78 79 80 81 82 83 84 85 86 87 88 89 90 91 92 93 94 95 96 97]
      | sbobj.Groups.Signals(32).YData = [0 0 0 0 0 1 1 1 1 1 1 1 1 2 2 2 2 2 2 2 2 2 2 2 3 3 3 3 3 3 3 3 3 3 3 3 3 3 3 3 4 4 4 4 4 4 4 4 4 4 4 4 4 4 4 4 5 5 5 5 5 5 5 5 5 5 5 5 5 5 5 5 6 6 6 6 6 6 6 6 6 6 6 6 6 6 6 6 6 6 6 6 6 6 6 6 6 6]
      | sbobj.Groups.Signals(33).Name = 'FW_manual'
      | sbobj.Groups.Signals(33).XData = [0 1 2 3 4 5 6 7 8 9 10 11 12 13 14 15 16 17 18 19 20 21 22 23 24 25 26 27 28 29 30 31 32 33 34 35 36 37 38 39 40 41 42 43 44 45 46 47 48 49 50 51 52 53 54 55 56 57 58 59 60 61 62 63 64 65 66 67 68 69 70 71 72 73 74 75 76 77 78 79 80 81 82 83 84 85 86 87 88 89 90 91 92 93 94 95 96 97]
      | sbobj.Groups.Signals(33).YData = [0 0 0 1 1 0 0 0 0 0 1 0 0 0 0 0 0 1 1 31 61 100 0 0 0 0 0 0 0 0 0 0 1 1 1 1 1 1 1 1 0 0 0 0 0 0 0 0 1 1 1 1 1 1 1 1 0 0 0 0 0 0 0 0 1 1 1 1 1 1 1 1 0 0 0 0 0 0 0 0 1 1 1 1 1 1 1 1 31 25 26 24 21 50 54 65 75 98]
      | sbobj.Groups.Signals(34).Name = 'WC_BackS'
      | sbobj.Groups.Signals(34).XData = [0 1 2 3 4 5 6 7 8 9 10 11 12 13 14 15 16 17 18 19 20 21 22 23 24 25 26 27 28 29 30 31 32 33 34 35 36 37 38 39 40 41 42 43 44 45 46 47 48 49 50 51 52 53 54 55 56 57 58 59 60 61 62 63 64 65 66 67 68 69 70 71 72 73 74 75 76 77 78 79 80 81 82 83 84 85 86 87 88 89 90 91 92 93 94 95 96 97]
      | sbobj.Groups.Signals(34).YData = [0 1 1 1 1 0 0 0 0 1 1 1 1 0 0 1 1 0 1 1 1 1 0 1 0 0 0 0 1 1 1 1 0 0 0 0 1 1 1 1 0 0 0 0 1 1 1 1 0 0 0 0 1 1 1 1 0 0 0 0 1 1 1 1 0 0 0 0 1 1 1 1 0 0 0 0 1 1 1 1 0 0 0 0 1 1 1 1 0 0 0 0 0 1 0 0 1 0]
      | sbobj.Groups.Signals(35).Name = 'WC_FrontS'
      | sbobj.Groups.Signals(35).XData = [0 1 2 3 4 5 6 7 8 9 10 11 12 13 14 15 16 17 18 19 20 21 22 23 24 25 26 27 28 29 30 31 32 33 34 35 36 37 38 39 40 41 42 43 44 45 46 47 48 49 50 51 52 53 54 55 56 57 58 59 60 61 62 63 64 65 66 67 68 69 70 71 72 73 74 75 76 77 78 79 80 81 82 83 84 85 86 87 88 89 90 91 92 93 94 95 96 97]
      | sbobj.Groups.Signals(35).YData = [0 0 0 1 1 1 1 1 1 0 1 1 1 1 1 0 0 1 1 1 1 1 1 0 0 0 1 1 0 0 1 1 0 0 1 1 0 0 1 1 0 0 1 1 0 0 1 1 0 0 1 1 0 0 1 1 0 0 1 1 0 0 1 1 0 0 1 1 0 0 1 1 0 0 1 1 0 0 1 1 0 0 1 1 0 0 1 1 1 0 1 1 1 1 1 1 1 0]
      | sbobj.Groups.Signals(36).Name = 'WC_Status'
      | sbobj.Groups.Signals(36).XData = [0 1 2 3 4 5 6 7 8 9 10 11 12 13 14 15 16 17 18 19 20 21 22 23 24 25 26 27 28 29 30 31 32 33 34 35 36 37 38 39 40 41 42 43 44 45 46 47 48 49 50 51 52 53 54 55 56 57 58 59 60 61 62 63 64 65 66 67 68 69 70 71 72 73 74 75 76 77 78 79 80 81 82 83 84 85 86 87 88 89 90 91 92 93 94 95 96 97]
      | sbobj.Groups.Signals(36).YData = [0 0 1 1 0 0 1 1 0 1 1 1 0 0 1 1 0 1 1 1 1 1 1 1 0 1 0 1 0 1 0 1 0 1 0 1 0 1 0 1 0 1 0 1 0 1 0 1 0 1 0 1 0 1 0 1 0 1 0 1 0 1 0 1 0 1 0 1 0 1 0 1 0 1 0 1 0 1 0 1 0 1 0 1 0 1 0 1 1 1 1 1 1 1 0 1 1 1]
      | sbobj.Groups.TimeRange = [0 97]
  Front_left_CP : Outport  Tag=STV Outport
  Right_left_CP : Outport  Tag=STV Outport  Port=2
  Right_right_CP : Outport  Tag=STV Outport  Port=3
  Driver_control : Outport  Tag=STV Outport  Port=4
  Front_left_DC : Outport  Tag=STV Outport  Port=5
  rear_left_DC : Outport  Tag=STV Outport  Port=6
  rear_right_DC : Outport  Tag=STV Outport  Port=7
  oject_detection_FL : Outport  Tag=STV Outport  Port=8
  Lock_Unlock : Outport  Tag=STV Outport  Port=9
  iginition : Outport  Tag=STV Outport  Port=10
  oject_detection_RL : Outport  Tag=STV Outport  Port=11
  oject_detection_RR : Outport  Tag=STV Outport  Port=12
  oject_detection_driver : Outport  Tag=STV Outport  Port=13
  ignition status : Outport  Tag=STV Outport  Port=14
  Door_1 : Outport  Tag=STV Outport  Port=15
  Door_2 : Outport  Tag=STV Outport  Port=16
  Door_3 : Outport  Tag=STV Outport  Port=17
  Door_4 : Outport  Tag=STV Outport  Port=18
  antilockleature : Outport  Tag=STV Outport  Port=19
  accln : Outport  Tag=STV Outport  Port=20
  BCM_Airbag_VehicleSpeed : Outport  Tag=STV Outport  Port=21
  BCM_Airbag_YawRate : Outport  Tag=STV Outport  Port=22
  BCM_Airbag_Air_ACC : Outport  Tag=STV Outport  Port=23
  BCM_Airbag_Driver_L : Outport  Tag=STV Outport  Port=24
  BCM_Airbag_L_Front_1 : Outport  Tag=STV Outport  Port=25
  BCM_Airbag_L_Rear_1 : Outport  Tag=STV Outport  Port=26
  BCM_Airbag_R_Rear_ : Outport  Tag=STV Outport  Port=27
  tier_pressure_1 : Outport  Tag=STV Outport  Port=28
  tier_pressure_2 : Outport  Tag=STV Outport  Port=29
  tier_pressure_3 : Outport  Tag=STV Outport  Port=30
  tier_pressure_4 : Outport  Tag=STV Outport  Port=31
  FW_Modes : Outport  Tag=STV Outport  Port=32
  FW_manual : Outport  Tag=STV Outport  Port=33
  WC_BackS : Outport  Tag=STV Outport  Port=34
  WC_FrontS : Outport  Tag=STV Outport  Port=35
  WC_Status : Outport  Tag=STV Outport  Port=36
  wires:
  Demux/1 -> Front_left_CP/1
  FromWs/1 -> Demux/1
  Demux/2 -> Right_left_CP/1
  Demux/3 -> Right_right_CP/1
  Demux/4 -> Driver_control/1
  Demux/5 -> Front_left_DC/1
  Demux/6 -> rear_left_DC/1
  Demux/7 -> rear_right_DC/1
  Demux/8 -> oject_detection_FL/1
  Demux/9 -> Lock_Unlock/1
  Demux/10 -> iginition/1
  Demux/11 -> oject_detection_RL/1
  Demux/12 -> oject_detection_RR/1
  Demux/13 -> oject_detection_driver/1
  Demux/14 -> ignition status/1
  Demux/15 -> Door_1/1
  Demux/16 -> Door_2/1
  Demux/17 -> Door_3/1
  Demux/18 -> Door_4/1
  Demux/19 -> antilockleature/1
  Demux/20 -> accln/1
  Demux/21 -> BCM_Airbag_VehicleSpeed/1
  Demux/22 -> BCM_Airbag_YawRate/1
  Demux/23 -> BCM_Airbag_Air_ACC/1
  Demux/24 -> BCM_Airbag_Driver_L/1
  Demux/25 -> BCM_Airbag_L_Front_1/1
  Demux/26 -> BCM_Airbag_L_Rear_1/1
  Demux/27 -> BCM_Airbag_R_Rear_/1
  Demux/28 -> tier_pressure_1/1
  Demux/29 -> tier_pressure_2/1
  Demux/30 -> tier_pressure_3/1
  Demux/31 -> tier_pressure_4/1
  Demux/32 -> FW_Modes/1
  Demux/33 -> FW_manual/1
  Demux/34 -> WC_BackS/1
  Demux/35 -> WC_FrontS/1
  Demux/36 -> WC_Status/1

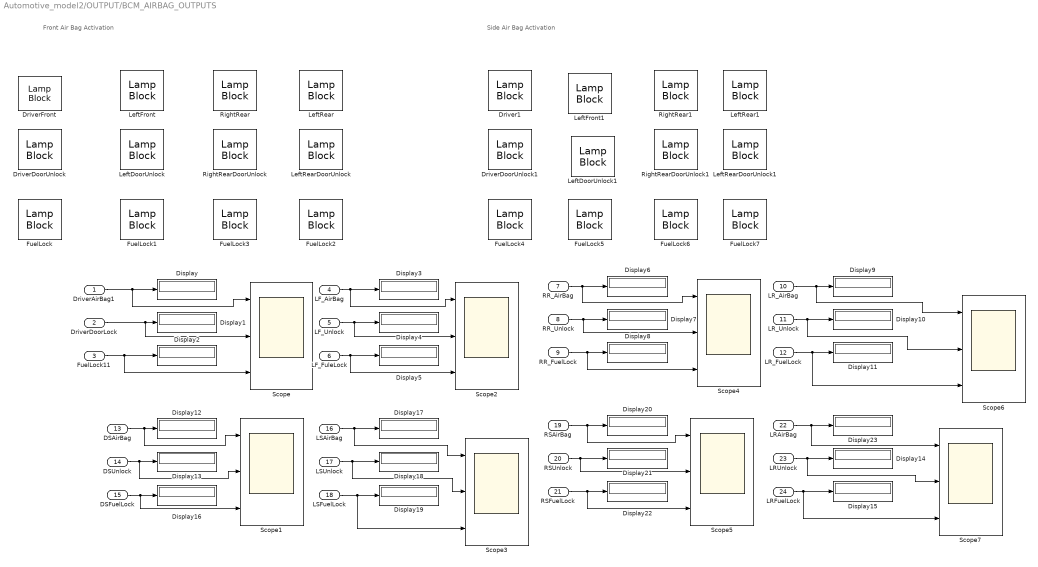
== system Automotive_model2/OUTPUT/BCM_AIRBAG_OUTPUTS ==
  note: Front Air Bag Activation
  note: Side Air Bag Activation
  DriverAirBag1 : Inport
  DriverDoorLock : Inport  Port=2
  FuelLock11 : Inport  Port=3
  LF_AirBag : Inport  Port=4
  LF_Unlock : Inport  Port=5
  LF_FuleLock : Inport  Port=6
  RR_AirBag : Inport  Port=7
  RR_Unlock : Inport  Port=8
  RR_FuelLock : Inport  Port=9
  LR_AirBag : Inport  Port=10
  LR_Unlock : Inport  Port=11
  LR_FuelLock : Inport  Port=12
  DSAirBag : Inport  Port=13
  DSUnlock : Inport  Port=14
  DSFuelLock : Inport  Port=15
  LSAirBag : Inport  Port=16
  LSUnlock : Inport  Port=17
  LSFuelLock : Inport  Port=18
  RSAirBag : Inport  Port=19
  RSUnlock : Inport  Port=20
  RSFuelLock : Inport  Port=21
  LRAirBag : Inport  Port=22
  LRUnlock : Inport  Port=23
  LRFuelLock : Inport  Port=24
  Display{,1..23} (24 alike) : Display
  Driver1 : LampBlock
  DriverDoorUnlock : LampBlock
  DriverDoorUnlock1 : LampBlock
  DriverFront : LampBlock
  FuelLock{,1..7} (8 alike) : LampBlock
  LeftDoorUnlock : LampBlock
  LeftDoorUnlock1 : LampBlock
  LeftFront : LampBlock
  LeftFront1 : LampBlock
  LeftRear : LampBlock
  LeftRear1 : LampBlock
  LeftRearDoorUnlock : LampBlock
  LeftRearDoorUnlock1 : LampBlock
  RightRear : LampBlock
  RightRear1 : LampBlock
  RightRearDoorUnlock : LampBlock
  RightRearDoorUnlock1 : LampBlock
  Scope{,1..7} (8 alike) : Scope  NumInputPorts=3
  wires:
  DriverAirBag1/1 -> Scope/1, Display/1
  FuelLock11/1 -> Scope/3, Display2/1
  LF_AirBag/1 -> Scope2/1, Display3/1
  LF_Unlock/1 -> Scope2/2, Display4/1
  RR_AirBag/1 -> Scope4/1, Display6/1
  RR_Unlock/1 -> Scope4/2, Display7/1
  RR_FuelLock/1 -> Scope4/3, Display8/1
  LR_AirBag/1 -> Scope6/1, Display9/1
  LR_Unlock/1 -> Scope6/2, Display10/1
  LR_FuelLock/1 -> Scope6/3, Display11/1
  DSFuelLock/1 -> Scope1/3, Display16/1
  LRAirBag/1 -> Scope7/1, Display23/1
  RSUnlock/1 -> Scope5/2, Display21/1
  RSAirBag/1 -> Scope5/1, Display20/1
  RSFuelLock/1 -> Scope5/3, Display22/1
  DSUnlock/1 -> Scope1/2, Display13/1
  LSUnlock/1 -> Scope3/2, Display18/1
  LRUnlock/1 -> Scope7/2, Display14/1
  LSFuelLock/1 -> Scope3/3, Display19/1
  LSAirBag/1 -> Scope3/1, Display17/1
  LRFuelLock/1 -> Scope7/3, Display15/1
  DSAirBag/1 -> Scope1/1, Display12/1
  DriverDoorLock/1 -> Scope/2, Display1/1
  LF_FuleLock/1 -> Scope2/3, Display5/1

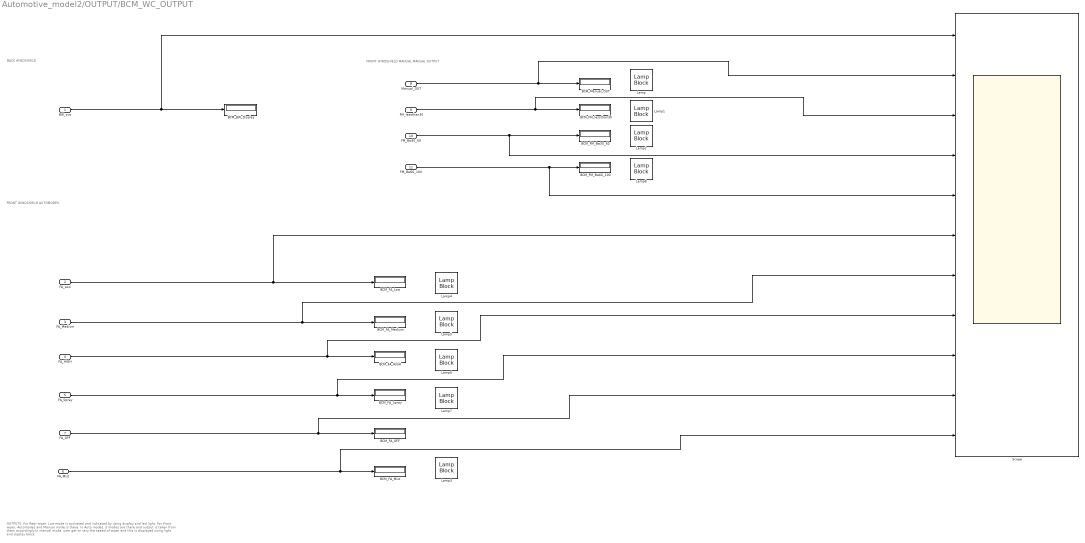
== system Automotive_model2/OUTPUT/BCM_WC_OUTPUT ==
  note: OUTPUTS:
      | For Rear wiper, Low mode is activated and indicated by using display and led light.
      | For Front wiper, Automodes and Manual mode is there.
      | In Auto modes, 5 modes are there and output is taken from them accordingly
      | In manual mode, user get to vary the speed of wiper and this is displayed using light and display block.
  note: BACK WINDSHIELD
  note: FRONT WINDSHIELD AUTOMODES
  note: FRONT WINDSHIELD MANUAL MANUAL OUTPUT
  BW_out : Inport
  FA_Low : Inport  Port=2
  FA_Medium : Inport  Port=3
  FA_HIGH : Inport  Port=4
  FA_Spray : Inport  Port=5
  FA_Mist : Inport  Port=6
  FA_OFF : Inport  Port=7
  Manual_OUT : Inport  Port=8
  FM_lessthan30 : Inport  Port=9
  FM_Bw30_60 : Inport  Port=10
  FM_Bw60_100 : Inport  Port=11
  BCM_BW_Display : Display
  BCM_FA_HIGH : Display
  BCM_FA_Low : Display
  BCM_FA_Medium : Display
  BCM_FA_Mist : Display
  BCM_FA_OFF : Display
  BCM_FA_Spray : Display
  BCM_FM_Bw30_60 : Display
  BCM_FM_Bw60_100 : Display
  BCM_FM_lessthan30 : Display
  BCM_Manual_OUT : Display
  Lamp{,1..8} (9 alike) : LampBlock
  Scope : Scope  NumInputPorts=11
  wires:
  BW_out/1 -> Scope/1, BCM_BW_Display/1
  FM_lessthan30/1 -> Scope/3, BCM_FM_lessthan30/1
  FM_Bw30_60/1 -> Scope/4, BCM_FM_Bw30_60/1
  FA_Low/1 -> Scope/6, BCM_FA_Low/1
  FA_Medium/1 -> Scope/7, BCM_FA_Medium/1
  FA_HIGH/1 -> Scope/8, BCM_FA_HIGH/1
  FA_Spray/1 -> Scope/9, BCM_FA_Spray/1
  FA_OFF/1 -> Scope/10, BCM_FA_OFF/1
  FA_Mist/1 -> Scope/11, BCM_FA_Mist/1
  Manual_OUT/1 -> Scope/2, BCM_Manual_OUT/1
  FM_Bw60_100/1 -> Scope/5, BCM_FM_Bw60_100/1

== system Automotive_model2/OUTPUT/Subsystem2 ==
  note: BCM_Door_system
  note: POWER_WINDOW_OP
  In1 : Inport
  In2 : Inport  Port=2
  In3 : Inport  Port=3
  In4 : Inport  Port=4
  In5 : Inport  Port=5
  In6 : Inport  Port=6
  In7 : Inport  Port=7
  In8 : Inport  Port=8
  Delay : Inport  Port=9
  Interior light : Inport  Port=10
  Automatic : Inport  Port=11
  Output_window_scope : Scope  NumInputPorts=8
  Scope3 : Scope  NumInputPorts=3
  wires:
  In2/1 -> Output_window_scope/2  "front_left_wind_pos"
  In1/1 -> Output_window_scope/1  "front_left_warn"
  In8/1 -> Output_window_scope/8  "driver_side_wind_pos"
  In5/1 -> Output_window_scope/5  "rear_right_warn"
  In3/1 -> Output_window_scope/3  "rear_left_warn"
  In4/1 -> Output_window_scope/4  "rear_left_wind_pos"
  In7/1 -> Output_window_scope/7  "driver_side_warn"
  In6/1 -> Output_window_scope/6  "rear_right_window_pos"
  Automatic/1 -> Scope3/1
  Delay/1 -> Scope3/2
  Interior light/1 -> Scope3/3

== system Automotive_model2/BCM_SAFETY_MODULE/BCM_AIRBAGSYSTEM/BCM_AB_CheckCrashType ==
  YawRate : Inport
  Air_ACC : Inport  Port=2
  Val_Side : Inport  Port=3
  AND : Logic  IconShape=distinctive  AllPortsSameDT=off  OutDataTypeStr=boolean
  AND1 : Logic  IconShape=distinctive  AllPortsSameDT=off  OutDataTypeStr=boolean
  ActivateAirBagSensor : MATLAB Function  TreatAsAtomicUnit=on
  CheckYawRateForFront : RelationalOperator  Operator===  OutDataTypeStr=boolean  RndMeth=Simplest
  CheckYawRateForSide : RelationalOperator  Operator===  OutDataTypeStr=boolean  RndMeth=Simplest
  Val_Front : Constant  Value=50
  Front_AirBag : Outport
  Side_AirBag : Outport  Port=2
  wires:
  CheckYawRateForSide/1 -> AND1/2
  ActivateAirBagSensor/1(AirBagSensor) -> AND1/1, AND/2
  CheckYawRateForFront/1 -> AND/1
  Air_ACC/1 -> ActivateAirBagSensor/1(SuddenDeceleration)
  Val_Side/1 -> CheckYawRateForSide/2
  YawRate/1 -> CheckYawRateForSide/1, CheckYawRateForFront/1
  Val_Front/1 -> CheckYawRateForFront/2
  AND1/1 -> Side_AirBag/1
  AND/1 -> Front_AirBag/1
